simulink model "Dec_10_updated_33_bus_system_2MW_DG"  (R2023a)
settings: Solver=FixedStepAuto  StartTime=0.0  StopTime=0.3  RelTol=1e-3  EnableMultiTasking=on
undefined symbols (not defined in the file or in its folder): D1, Delta, DiscIntNeverNeededParam, Ts, Ts_Power
libraries: spsSeriesRLCBranchLib x42, spsThreePhaseVIMeasurementLib x35, spsThreePhaseSeriesRLCBranchLib x33, spsLoadFlowBusLib x33, spsThreePhaseParallelRLCLoadLib x31, simulink x8, spsMeanLib x5, spsFirstOrderFilterLib x4, spsStairGeneratorLib x3, spsBoostConverterLib x2, spsPowerPositiveSequenceLib x2, spsabctodq0Lib x2
(part 1 of 3)
settings Model: ExtModeTrigDuration=2  Creator=Archana  LastModifiedBy=praka
settings SolverCC: AutoInsertRateTranBlk=on
settings OptimizationCC: EnhancedBackFolding=on  PassReuseOutputArgsAs=Individual arguments  ZeroExternalMemoryAtStartup=off  ZeroInternalMemoryAtStartup=off  MaxStackSize=64  OptimizeBlockOrder=speed  DifferentSizesBufferReuse=on  OptimizationCustomize=off  EfficientTunableParamExpr=on
settings DebuggingCC: ParameterTunabilityLossMsg=error
settings HardwareCC: ProdBitPerPointer=32  ProdBitPerSizeT=32  ProdBitPerPtrDiffT=32  ProdLargestAtomicInteger=Long  ProdLargestAtomicFloat=Double  ProdWordSize=32  ProdHWDeviceType=ARM Compatible->ARM Cortex
settings SFSimCC: MATLABDynamicMemAlloc=off
settings RTWCC: Description=Embedded Coder  SystemTargetFile=ert.tlc  HardwareBoard=ESP32-WROVER(Arduino Compatible)  TLCOptions="-aInlineSetEventsForThisBaseRateFcn=TLC_FALSE -aSuppressMultiTaskScheduler=TLC_FALSE  -aRateBasedStepFcn=0"  TemplateMakefile=ert_default_tmf  Toolchain=ESP32  BuildConfiguration=Faster Runs
settings CodeAppCC: ForceParamTrailComments=on  IgnoreCustomStorageClasses=off  OperatorAnnotations=on  SimulinkDataObjDesc=on  SFDataObjDesc=on  InsertBlockDesc=on
settings ERTTargetCC: SupportContinuousTime=on  SupportVariableSizeSignals=on  ExtModeTransport=3  ExtModeStaticAlloc=on  ExtModeAutomaticAllocSize=off  ExtModeStaticAllocSize=65536  ExtModeMexFile=ext_xcp  ExtModeIntrfLevel=Level2 - Open

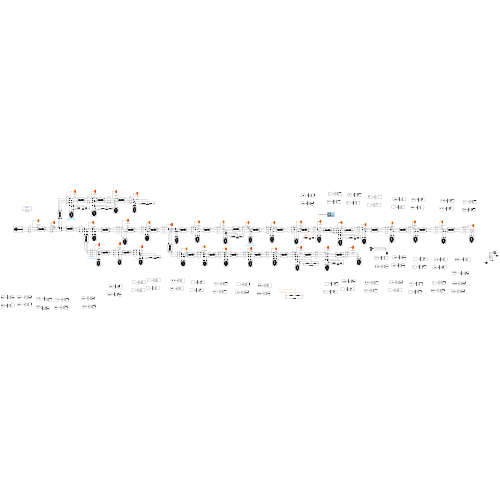
[thumbnail: Simulink's stored preview of the top-level diagram]
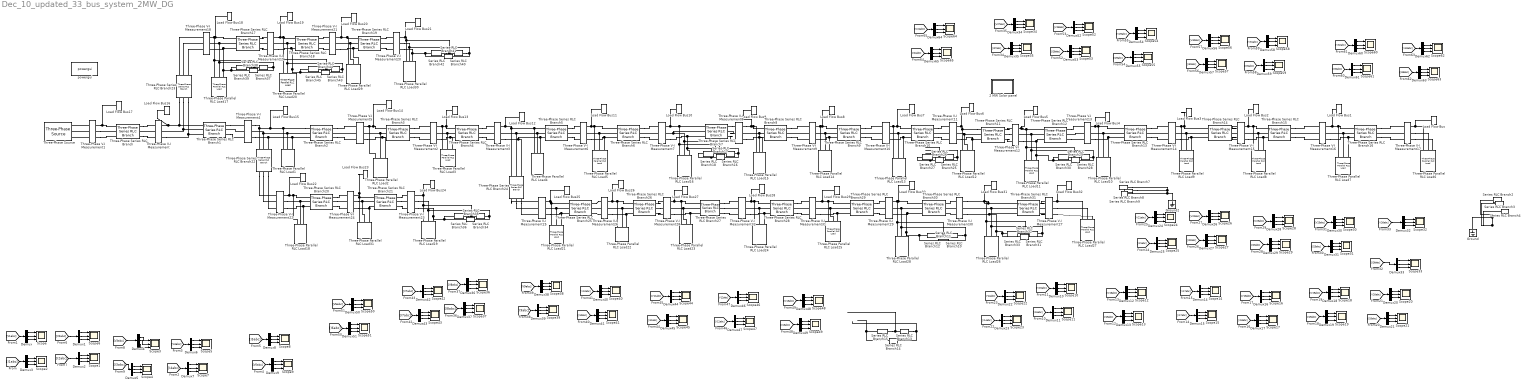
== system Dec_10_updated_33_bus_system_2MW_DG ==
  2 MW Solar panel : Subsystem
  Demux{,1..65} (66 alike) : Demux  Outputs=3
  Ground : spsGroundLib/Ground  LConnTagsString=a
  Ground2 : spsGroundLib/Ground  LConnTagsString=a
  Load Flow Bus : spsLoadFlowBusLib/Load Flow Bus  LConnTagsString=a  Phases=single  Connectors=on one side  ID=18  Vbase=12.66e3  Vref=1  Vangle=0  VLF=1  VLFb=1  VLFc=1  angleLF=0  angleLFb=0  angleLFc=0
  Load Flow Bus1 : spsLoadFlowBusLib/Load Flow Bus  LConnTagsString=a  Phases=single  Connectors=on one side  ID=17  Vbase=12.66e3  Vref=1  Vangle=0  VLF=1  VLFb=1  VLFc=1  angleLF=0  angleLFb=0  angleLFc=0
  Load Flow Bus10 : spsLoadFlowBusLib/Load Flow Bus  LConnTagsString=a  Phases=single  Connectors=on one side  ID=8  Vbase=12.66e3  Vref=1  Vangle=0  VLF=1  VLFb=1  VLFc=1  angleLF=0  angleLFb=0  angleLFc=0
  Load Flow Bus11 : spsLoadFlowBusLib/Load Flow Bus  LConnTagsString=a  Phases=single  Connectors=on one side  ID=7  Vbase=12.66e3  Vref=1  Vangle=0  VLF=1  VLFb=1  VLFc=1  angleLF=0  angleLFb=0  angleLFc=0
  Load Flow Bus12 : spsLoadFlowBusLib/Load Flow Bus  LConnTagsString=a  Phases=single  Connectors=on one side  ID=6  Vbase=12.66e3  Vref=1  Vangle=0  VLF=1  VLFb=1  VLFc=1  angleLF=0  angleLFb=0  angleLFc=0
  Load Flow Bus13 : spsLoadFlowBusLib/Load Flow Bus  LConnTagsString=a  Phases=single  Connectors=on one side  ID=5  Vbase=12.66e3  Vref=1  Vangle=0  VLF=1  VLFb=1  VLFc=1  angleLF=0  angleLFb=0  angleLFc=0
  Load Flow Bus14 : spsLoadFlowBusLib/Load Flow Bus  LConnTagsString=a  Phases=single  Connectors=on one side  ID=4  Vbase=12.66e3  Vref=1  Vangle=0  VLF=1  VLFb=1  VLFc=1  angleLF=0  angleLFb=0  angleLFc=0
  Load Flow Bus15 : spsLoadFlowBusLib/Load Flow Bus  LConnTagsString=a  Phases=single  Connectors=on one side  ID=3  Vbase=12.66e3  Vref=1  Vangle=0  VLF=1  VLFb=1  VLFc=1  angleLF=0  angleLFb=0  angleLFc=0
  Load Flow Bus16 : spsLoadFlowBusLib/Load Flow Bus  LConnTagsString=a  Phases=single  Connectors=on one side  ID=2  Vbase=12.66e3  Vref=1  Vangle=0  VLF=1  VLFb=1  VLFc=1  angleLF=0  angleLFb=0  angleLFc=0
  Load Flow Bus17 : spsLoadFlowBusLib/Load Flow Bus  LConnTagsString=a  Phases=single  Connectors=on one side  ID=1  Vbase=12.66e3  Vref=1.05  Vangle=0  VLF=1  VLFb=1  VLFc=1  angleLF=0  angleLFb=0  angleLFc=0
  Load Flow Bus18 : spsLoadFlowBusLib/Load Flow Bus  LConnTagsString=a  Phases=single  Connectors=on one side  ID=19  Vbase=12.66e3  Vref=1  Vangle=0  VLF=1  VLFb=1  VLFc=1  angleLF=0  angleLFb=0  angleLFc=0
  Load Flow Bus19 : spsLoadFlowBusLib/Load Flow Bus  LConnTagsString=a  Phases=single  Connectors=on one side  ID=20  Vbase=12.66e3  Vref=1  Vangle=0  VLF=1  VLFb=1  VLFc=1  angleLF=0  angleLFb=0  angleLFc=0
  Load Flow Bus2 : spsLoadFlowBusLib/Load Flow Bus  LConnTagsString=a  Phases=single  Connectors=on one side  ID=16  Vbase=12.66e3  Vref=1  Vangle=0  VLF=1  VLFb=1  VLFc=1  angleLF=0  angleLFb=0  angleLFc=0
  Load Flow Bus20 : spsLoadFlowBusLib/Load Flow Bus  LConnTagsString=a  Phases=single  Connectors=on one side  ID=21  Vbase=12.66e3  Vref=1  Vangle=0  VLF=1  VLFb=1  VLFc=1  angleLF=0  angleLFb=0  angleLFc=0
  Load Flow Bus21 : spsLoadFlowBusLib/Load Flow Bus  LConnTagsString=a  Phases=single  Connectors=on one side  ID=22  Vbase=12.66e3  Vref=1  Vangle=0  VLF=1  VLFb=1  VLFc=1  angleLF=0  angleLFb=0  angleLFc=0
  Load Flow Bus22 : spsLoadFlowBusLib/Load Flow Bus  LConnTagsString=a  Phases=single  Connectors=on one side  ID=23  Vbase=33e3  Vref=1  Vangle=0  VLF=1  VLFb=1  VLFc=1  angleLF=0  angleLFb=0  angleLFc=0
  Load Flow Bus23 : spsLoadFlowBusLib/Load Flow Bus  LConnTagsString=a  Phases=single  Connectors=on one side  ID=24  Vbase=33e3  Vref=1  Vangle=0  VLF=1  VLFb=1  VLFc=1  angleLF=0  angleLFb=0  angleLFc=0
  Load Flow Bus24 : spsLoadFlowBusLib/Load Flow Bus  LConnTagsString=a  Phases=single  Connectors=on one side  ID=25  Vbase=33e3  Vref=1  Vangle=0  VLF=1  VLFb=1  VLFc=1  angleLF=0  angleLFb=0  angleLFc=0
  Load Flow Bus25 : spsLoadFlowBusLib/Load Flow Bus  LConnTagsString=a  Phases=single  Connectors=on one side  ID=26  Vbase=12.66e3  Vref=1  Vangle=0  VLF=1  VLFb=1  VLFc=1  angleLF=0  angleLFb=0  angleLFc=0
  Load Flow Bus26 : spsLoadFlowBusLib/Load Flow Bus  LConnTagsString=a  Phases=single  Connectors=on one side  ID=27  Vbase=12.66e3  Vref=1  Vangle=0  VLF=1  VLFb=1  VLFc=1  angleLF=0  angleLFb=0  angleLFc=0
  Load Flow Bus27 : spsLoadFlowBusLib/Load Flow Bus  LConnTagsString=a  Phases=single  Connectors=on one side  ID=28  Vbase=12.66e3  Vref=1  Vangle=0  VLF=1  VLFb=1  VLFc=1  angleLF=0  angleLFb=0  angleLFc=0
  Load Flow Bus28 : spsLoadFlowBusLib/Load Flow Bus  LConnTagsString=a  Phases=single  Connectors=on one side  ID=29  Vbase=12.66e3  Vref=1  Vangle=0  VLF=1  VLFb=1  VLFc=1  angleLF=0  angleLFb=0  angleLFc=0
  Load Flow Bus29 : spsLoadFlowBusLib/Load Flow Bus  LConnTagsString=a  Phases=single  Connectors=on one side  ID=30  Vbase=12.66e3  Vref=1  Vangle=0  VLF=1  VLFb=1  VLFc=1  angleLF=0  angleLFb=0  angleLFc=0
  Load Flow Bus3 : spsLoadFlowBusLib/Load Flow Bus  LConnTagsString=a  Phases=single  Connectors=on one side  ID=15  Vbase=12.66e3  Vref=1  Vangle=0  VLF=1  VLFb=1  VLFc=1  angleLF=0  angleLFb=0  angleLFc=0
  Load Flow Bus30 : spsLoadFlowBusLib/Load Flow Bus  LConnTagsString=a  Phases=single  Connectors=on one side  ID=31  Vbase=12.66e3  Vref=1  Vangle=0  VLF=1  VLFb=1  VLFc=1  angleLF=0  angleLFb=0  angleLFc=0
  Load Flow Bus31 : spsLoadFlowBusLib/Load Flow Bus  LConnTagsString=a  Phases=single  Connectors=on one side  ID=32  Vbase=12.66e3  Vref=1  Vangle=0  VLF=1  VLFb=1  VLFc=1  angleLF=0  angleLFb=0  angleLFc=0
  Load Flow Bus32 : spsLoadFlowBusLib/Load Flow Bus  LConnTagsString=a  Phases=single  Connectors=on one side  ID=33  Vbase=12.66e3  Vref=1  Vangle=0  VLF=1  VLFb=1  VLFc=1  angleLF=0  angleLFb=0  angleLFc=0
  Load Flow Bus4 : spsLoadFlowBusLib/Load Flow Bus  LConnTagsString=a  Phases=single  Connectors=on one side  ID=14  Vbase=12.66e3  Vref=1  Vangle=0  VLF=1  VLFb=1  VLFc=1  angleLF=0  angleLFb=0  angleLFc=0
  Load Flow Bus5 : spsLoadFlowBusLib/Load Flow Bus  LConnTagsString=a  Phases=single  Connectors=on one side  ID=13  Vbase=12.66e3  Vref=1  Vangle=0  VLF=1  VLFb=1  VLFc=1  angleLF=0  angleLFb=0  angleLFc=0
  Load Flow Bus6 : spsLoadFlowBusLib/Load Flow Bus  LConnTagsString=a  Phases=single  Connectors=on one side  ID=12  Vbase=12.66e3  Vref=1  Vangle=0  VLF=1  VLFb=1  VLFc=1  angleLF=0  angleLFb=0  angleLFc=0
  Load Flow Bus7 : spsLoadFlowBusLib/Load Flow Bus  LConnTagsString=a  Phases=single  Connectors=on one side  ID=11  Vbase=12.66e3  Vref=1  Vangle=0  VLF=1  VLFb=1  VLFc=1  angleLF=0  angleLFb=0  angleLFc=0
  Load Flow Bus8 : spsLoadFlowBusLib/Load Flow Bus  LConnTagsString=a  Phases=single  Connectors=on one side  ID=10  Vbase=12.66e3  Vref=1  Vangle=0  VLF=1  VLFb=1  VLFc=1  angleLF=0  angleLFb=0  angleLFc=0
  Load Flow Bus9 : spsLoadFlowBusLib/Load Flow Bus  LConnTagsString=a  Phases=single  Connectors=on one side  ID=9  Vbase=12.66e3  Vref=1  Vangle=0  VLF=1  VLFb=1  VLFc=1  angleLF=0  angleLFb=0  angleLFc=0
  Scope{,1..65} (66 alike) : Scope  NumInputPorts=3
  Series RLC Branch10 : spsSeriesRLCBranchLib/Series RLC Branch  LConnTagsString=__new0  RConnTagsString=__new0  BranchType=C  Resistance=1  Inductance=0  SetiL0=off  InitialCurrent=0  Capacitance=4.53e-6  Setx0=off  InitialVoltage=0  Measurements=None
  Series RLC Branch11 : spsSeriesRLCBranchLib/Series RLC Branch  LConnTagsString=__new0  RConnTagsString=__new0  BranchType=C  Resistance=1  Inductance=0  SetiL0=off  InitialCurrent=0  Capacitance=4.53e-6  Setx0=off  InitialVoltage=0  Measurements=None
  Series RLC Branch12 : spsSeriesRLCBranchLib/Series RLC Branch  LConnTagsString=__new0  RConnTagsString=__new0  BranchType=C  Resistance=1  Inductance=0  SetiL0=off  InitialCurrent=0  Capacitance=4.53e-6  Setx0=off  InitialVoltage=0  Measurements=None
  Series RLC Branch13 : spsSeriesRLCBranchLib/Series RLC Branch  LConnTagsString=__new0  RConnTagsString=__new0  BranchType=C  Resistance=1  Inductance=0  SetiL0=off  InitialCurrent=0  Capacitance=0.144e-6  Setx0=off  InitialVoltage=0  Measurements=None
  Series RLC Branch14 : spsSeriesRLCBranchLib/Series RLC Branch  LConnTagsString=__new0  RConnTagsString=__new0  BranchType=C  Resistance=1  Inductance=0  SetiL0=off  InitialCurrent=0  Capacitance=0.144e-6  Setx0=off  InitialVoltage=0  Measurements=None
  Series RLC Branch15 : spsSeriesRLCBranchLib/Series RLC Branch  LConnTagsString=__new0  RConnTagsString=__new0  BranchType=C  Resistance=1  Inductance=0  SetiL0=off  InitialCurrent=0  Capacitance=0.144e-6  Setx0=off  InitialVoltage=0  Measurements=None
  Series RLC Branch16 : spsSeriesRLCBranchLib/Series RLC Branch  LConnTagsString=__new0  RConnTagsString=__new0  BranchType=C  Resistance=1  Inductance=0  SetiL0=off  InitialCurrent=0  Capacitance=1.44e-6  Setx0=off  InitialVoltage=0  Measurements=None
  Series RLC Branch17 : spsSeriesRLCBranchLib/Series RLC Branch  LConnTagsString=__new0  RConnTagsString=__new0  BranchType=C  Resistance=1  Inductance=0  SetiL0=off  InitialCurrent=0  Capacitance=1.44e-6  Setx0=off  InitialVoltage=0  Measurements=None
  Series RLC Branch18 : spsSeriesRLCBranchLib/Series RLC Branch  LConnTagsString=__new0  RConnTagsString=__new0  BranchType=C  Resistance=1  Inductance=0  SetiL0=off  InitialCurrent=0  Capacitance=1.44e-6  Setx0=off  InitialVoltage=0  Measurements=None
  Series RLC Branch2 : spsSeriesRLCBranchLib/Series RLC Branch  LConnTagsString=__new0  RConnTagsString=__new0  BranchType=C  Resistance=1  Inductance=0  SetiL0=off  InitialCurrent=0  Capacitance=3.26e-6  Setx0=off  InitialVoltage=0  Measurements=None
  Series RLC Branch25 : spsSeriesRLCBranchLib/Series RLC Branch  LConnTagsString=__new0  RConnTagsString=__new0  BranchType=C  Resistance=1  Inductance=0  SetiL0=off  InitialCurrent=0  Capacitance=0.755e-6  Setx0=off  InitialVoltage=0  Measurements=None
  Series RLC Branch26 : spsSeriesRLCBranchLib/Series RLC Branch  LConnTagsString=__new0  RConnTagsString=__new0  BranchType=C  Resistance=1  Inductance=0  SetiL0=off  InitialCurrent=0  Capacitance=0.755e-6  Setx0=off  InitialVoltage=0  Measurements=None
  Series RLC Branch27 : spsSeriesRLCBranchLib/Series RLC Branch  LConnTagsString=__new0  RConnTagsString=__new0  BranchType=C  Resistance=1  Inductance=0  SetiL0=off  InitialCurrent=0  Capacitance=0.755e-6  Setx0=off  InitialVoltage=0  Measurements=None
  Series RLC Branch28 : spsSeriesRLCBranchLib/Series RLC Branch  LConnTagsString=__new0  RConnTagsString=__new0  BranchType=C  Resistance=1  Inductance=0  SetiL0=off  InitialCurrent=0  Capacitance=0.594e-6  Setx0=off  InitialVoltage=0  Measurements=None
  Series RLC Branch29 : spsSeriesRLCBranchLib/Series RLC Branch  LConnTagsString=__new0  RConnTagsString=__new0  BranchType=C  Resistance=1  Inductance=0  SetiL0=off  InitialCurrent=0  Capacitance=0.594e-6  Setx0=off  InitialVoltage=0  Measurements=None
  Series RLC Branch3 : spsSeriesRLCBranchLib/Series RLC Branch  LConnTagsString=__new0  RConnTagsString=__new0  BranchType=C  Resistance=1  Inductance=0  SetiL0=off  InitialCurrent=0  Capacitance=3.26e-6  Setx0=off  InitialVoltage=0  Measurements=None
  Series RLC Branch30 : spsSeriesRLCBranchLib/Series RLC Branch  LConnTagsString=__new0  RConnTagsString=__new0  BranchType=C  Resistance=1  Inductance=0  SetiL0=off  InitialCurrent=0  Capacitance=0.594e-6  Setx0=off  InitialVoltage=0  Measurements=None
  Series RLC Branch31 : spsSeriesRLCBranchLib/Series RLC Branch  LConnTagsString=__new0  RConnTagsString=__new0  BranchType=C  Resistance=1  Inductance=0  SetiL0=off  InitialCurrent=0  Capacitance=0.472e-6  Setx0=off  InitialVoltage=0  Measurements=None
  Series RLC Branch32 : spsSeriesRLCBranchLib/Series RLC Branch  LConnTagsString=__new0  RConnTagsString=__new0  BranchType=C  Resistance=1  Inductance=0  SetiL0=off  InitialCurrent=0  Capacitance=0.472e-6  Setx0=off  InitialVoltage=0  Measurements=None
  Series RLC Branch33 : spsSeriesRLCBranchLib/Series RLC Branch  LConnTagsString=__new0  RConnTagsString=__new0  BranchType=C  Resistance=1  Inductance=0  SetiL0=off  InitialCurrent=0  Capacitance=0.472e-6  Setx0=off  InitialVoltage=0  Measurements=None
  Series RLC Branch34 : spsSeriesRLCBranchLib/Series RLC Branch  LConnTagsString=__new0  RConnTagsString=__new0  BranchType=C  Resistance=1  Inductance=0  SetiL0=off  InitialCurrent=0  Capacitance=0.614e-6  Setx0=off  InitialVoltage=0  Measurements=None
  Series RLC Branch35 : spsSeriesRLCBranchLib/Series RLC Branch  LConnTagsString=__new0  RConnTagsString=__new0  BranchType=C  Resistance=1  Inductance=0  SetiL0=off  InitialCurrent=0  Capacitance=0.614e-6  Setx0=off  InitialVoltage=0  Measurements=None
  Series RLC Branch36 : spsSeriesRLCBranchLib/Series RLC Branch  LConnTagsString=__new0  RConnTagsString=__new0  BranchType=C  Resistance=1  Inductance=0  SetiL0=off  InitialCurrent=0  Capacitance=0.614e-6  Setx0=off  InitialVoltage=0  Measurements=None
  Series RLC Branch37 : spsSeriesRLCBranchLib/Series RLC Branch  LConnTagsString=__new0  RConnTagsString=__new0  BranchType=C  Resistance=1  Inductance=0  SetiL0=off  InitialCurrent=0  Capacitance=0.434e-6  Setx0=off  InitialVoltage=0  Measurements=None
  Series RLC Branch38 : spsSeriesRLCBranchLib/Series RLC Branch  LConnTagsString=__new0  RConnTagsString=__new0  BranchType=C  Resistance=1  Inductance=0  SetiL0=off  InitialCurrent=0  Capacitance=0.434e-6  Setx0=off  InitialVoltage=0  Measurements=None
  Series RLC Branch39 : spsSeriesRLCBranchLib/Series RLC Branch  LConnTagsString=__new0  RConnTagsString=__new0  BranchType=C  Resistance=1  Inductance=0  SetiL0=off  InitialCurrent=0  Capacitance=0.434e-6  Setx0=off  InitialVoltage=0  Measurements=None
  Series RLC Branch4 : spsSeriesRLCBranchLib/Series RLC Branch  LConnTagsString=__new0  RConnTagsString=__new0  BranchType=C  Resistance=1  Inductance=0  SetiL0=off  InitialCurrent=0  Capacitance=3.26e-6  Setx0=off  InitialVoltage=0  Measurements=None
  Series RLC Branch40 : spsSeriesRLCBranchLib/Series RLC Branch  LConnTagsString=__new0  RConnTagsString=__new0  BranchType=C  Resistance=1  Inductance=0  SetiL0=off  InitialCurrent=0  Capacitance=0.107e-6  Setx0=off  InitialVoltage=0  Measurements=None
  Series RLC Branch41 : spsSeriesRLCBranchLib/Series RLC Branch  LConnTagsString=__new0  RConnTagsString=__new0  BranchType=C  Resistance=1  Inductance=0  SetiL0=off  InitialCurrent=0  Capacitance=0.107e-6  Setx0=off  InitialVoltage=0  Measurements=None
  Series RLC Branch42 : spsSeriesRLCBranchLib/Series RLC Branch  LConnTagsString=__new0  RConnTagsString=__new0  BranchType=C  Resistance=1  Inductance=0  SetiL0=off  InitialCurrent=0  Capacitance=0.107e-6  Setx0=off  InitialVoltage=0  Measurements=None
  Series RLC Branch43 : spsSeriesRLCBranchLib/Series RLC Branch  LConnTagsString=__new0  RConnTagsString=__new0  BranchType=C  Resistance=1  Inductance=0  SetiL0=off  InitialCurrent=0  Capacitance=0.322e-6  Setx0=off  InitialVoltage=0  Measurements=None
  Series RLC Branch44 : spsSeriesRLCBranchLib/Series RLC Branch  LConnTagsString=__new0  RConnTagsString=__new0  BranchType=C  Resistance=1  Inductance=0  SetiL0=off  InitialCurrent=0  Capacitance=0.322e-6  Setx0=off  InitialVoltage=0  Measurements=None
  Series RLC Branch45 : spsSeriesRLCBranchLib/Series RLC Branch  LConnTagsString=__new0  RConnTagsString=__new0  BranchType=C  Resistance=1  Inductance=0  SetiL0=off  InitialCurrent=0  Capacitance=0.322e-6  Setx0=off  InitialVoltage=0  Measurements=None
  Series RLC Branch7 : spsSeriesRLCBranchLib/Series RLC Branch  LConnTagsString=__new0  RConnTagsString=__new0  BranchType=C  Resistance=1  Inductance=0  SetiL0=off  InitialCurrent=0  Capacitance=36.8e-6  Setx0=off  InitialVoltage=0  Measurements=None
  Series RLC Branch8 : spsSeriesRLCBranchLib/Series RLC Branch  LConnTagsString=__new0  RConnTagsString=__new0  BranchType=C  Resistance=1  Inductance=0  SetiL0=off  InitialCurrent=0  Capacitance=36.8e-6  Setx0=off  InitialVoltage=0  Measurements=None
  Series RLC Branch9 : spsSeriesRLCBranchLib/Series RLC Branch  LConnTagsString=__new0  RConnTagsString=__new0  BranchType=C  Resistance=1  Inductance=0  SetiL0=off  InitialCurrent=0  Capacitance=36.8e-6  Setx0=off  InitialVoltage=0  Measurements=None
  Three-Phase Parallel RLC Load1 : spsThreePhaseParallelRLCLoadLib/Three-Phase Parallel RLC Load  LConnTagsString=A|B|C  Configuration=Y (grounded)  NominalVoltage=12.66e3  Vabc=[1e3 1e3 1e3]  Vabcp=[1e3 1e3 1e3]  NominalFrequency=50  UnbalancedPower=off  ActivePower=100e3  InductivePower=60e3  CapacitivePower=0  Pabc=[10e3 9e3 11e3]  QLabc=[100 90 110]  QCabc=[100 90 110]  Pabcp=[10e3 9e3 11e3]  QLabcp=[100 90 110]  QCabcp=[100 90 110]  Measurements=None  LoadType=constant PQ
  Three-Phase Parallel RLC Load10 : spsThreePhaseParallelRLCLoadLib/Three-Phase Parallel RLC Load  LConnTagsString=A|B|C  Configuration=Y (grounded)  NominalVoltage=12.66e3  Vabc=[1e3 1e3 1e3]  Vabcp=[1e3 1e3 1e3]  NominalFrequency=50  UnbalancedPower=off  ActivePower=60e3  InductivePower=35e3  CapacitivePower=0  Pabc=[10e3 9e3 11e3]  QLabc=[100 90 110]  QCabc=[100 90 110]  Pabcp=[10e3 9e3 11e3]  QLabcp=[100 90 110]  QCabcp=[100 90 110]  Measurements=None  LoadType=constant PQ
  Three-Phase Parallel RLC Load11 : spsThreePhaseParallelRLCLoadLib/Three-Phase Parallel RLC Load  LConnTagsString=A|B|C  Configuration=Y (grounded)  NominalVoltage=12.66e3  Vabc=[1e3 1e3 1e3]  Vabcp=[1e3 1e3 1e3]  NominalFrequency=50  UnbalancedPower=off  ActivePower=60e3  InductivePower=35e3  CapacitivePower=0  Pabc=[10e3 9e3 11e3]  QLabc=[100 90 110]  QCabc=[100 90 110]  Pabcp=[10e3 9e3 11e3]  QLabcp=[100 90 110]  QCabcp=[100 90 110]  Measurements=None  LoadType=constant PQ
  Three-Phase Parallel RLC Load12 : spsThreePhaseParallelRLCLoadLib/Three-Phase Parallel RLC Load  LConnTagsString=A|B|C  Configuration=Y (grounded)  NominalVoltage=12.66e3  Vabc=[1e3 1e3 1e3]  Vabcp=[1e3 1e3 1e3]  NominalFrequency=50  UnbalancedPower=off  ActivePower=45e3  InductivePower=30e3  CapacitivePower=0  Pabc=[10e3 9e3 11e3]  QLabc=[100 90 110]  QCabc=[100 90 110]  Pabcp=[10e3 9e3 11e3]  QLabcp=[100 90 110]  QCabcp=[100 90 110]  Measurements=None  LoadType=constant PQ
  Three-Phase Parallel RLC Load{5..7,13..14,24} (6 alike) : spsThreePhaseParallelRLCLoadLib/Three-Phase Parallel RLC Load  LConnTagsString=A|B|C  Configuration=Y (grounded)  NominalVoltage=12.66e3  Vabc=[1e3 1e3 1e3]  Vabcp=[1e3 1e3 1e3]  NominalFrequency=50  UnbalancedPower=off  ActivePower=60e3  InductivePower=20e3  CapacitivePower=0  Pabc=[10e3 9e3 11e3]  QLabc=[100 90 110]  QCabc=[100 90 110]  Pabcp=[10e3 9e3 11e3]  QLabcp=[100 90 110]  QCabcp=[100 90 110]  Measurements=None  LoadType=constant PQ
  Three-Phase Parallel RLC Load15 : spsThreePhaseParallelRLCLoadLib/Three-Phase Parallel RLC Load  LConnTagsString=A|B|C  Configuration=Y (grounded)  NominalVoltage=12.66e3  Vabc=[1e3 1e3 1e3]  Vabcp=[1e3 1e3 1e3]  NominalFrequency=50  UnbalancedPower=off  ActivePower=200e3  InductivePower=100e3  CapacitivePower=0  Pabc=[10e3 9e3 11e3]  QLabc=[100 90 110]  QCabc=[100 90 110]  Pabcp=[10e3 9e3 11e3]  QLabcp=[100 90 110]  QCabcp=[100 90 110]  Measurements=None  LoadType=constant PQ
  Three-Phase Parallel RLC Load16 : spsThreePhaseParallelRLCLoadLib/Three-Phase Parallel RLC Load  LConnTagsString=A|B|C  Configuration=Y (grounded)  NominalVoltage=12.66e3  Vabc=[1e3 1e3 1e3]  Vabcp=[1e3 1e3 1e3]  NominalFrequency=50  UnbalancedPower=off  ActivePower=200e3  InductivePower=100e3  CapacitivePower=0  Pabc=[10e3 9e3 11e3]  QLabc=[100 90 110]  QCabc=[100 90 110]  Pabcp=[10e3 9e3 11e3]  QLabcp=[100 90 110]  QCabcp=[100 90 110]  Measurements=None  LoadType=constant PQ
  Three-Phase Parallel RLC Load{2,17..18,20,29..30} (6 alike) : spsThreePhaseParallelRLCLoadLib/Three-Phase Parallel RLC Load  LConnTagsString=A|B|C  Configuration=Y (grounded)  NominalVoltage=12.66e3  Vabc=[1e3 1e3 1e3]  Vabcp=[1e3 1e3 1e3]  NominalFrequency=50  UnbalancedPower=off  ActivePower=90e3  InductivePower=40e3  CapacitivePower=0  Pabc=[10e3 9e3 11e3]  QLabc=[100 90 110]  QCabc=[100 90 110]  Pabcp=[10e3 9e3 11e3]  QLabcp=[100 90 110]  QCabcp=[100 90 110]  Measurements=None  LoadType=constant PQ
  Three-Phase Parallel RLC Load19 : spsThreePhaseParallelRLCLoadLib/Three-Phase Parallel RLC Load  LConnTagsString=A|B|C  Configuration=Y (grounded)  NominalVoltage=12.66e3  Vabc=[1e3 1e3 1e3]  Vabcp=[1e3 1e3 1e3]  NominalFrequency=50  UnbalancedPower=off  ActivePower=420e3  InductivePower=200e3  CapacitivePower=0  Pabc=[10e3 9e3 11e3]  QLabc=[100 90 110]  QCabc=[100 90 110]  Pabcp=[10e3 9e3 11e3]  QLabcp=[100 90 110]  QCabcp=[100 90 110]  Measurements=None  LoadType=constant PQ
  Three-Phase Parallel RLC Load21 : spsThreePhaseParallelRLCLoadLib/Three-Phase Parallel RLC Load  LConnTagsString=A|B|C  Configuration=Y (grounded)  NominalVoltage=12.66e3  Vabc=[1e3 1e3 1e3]  Vabcp=[1e3 1e3 1e3]  NominalFrequency=50  UnbalancedPower=off  ActivePower=420e3  InductivePower=200e3  CapacitivePower=0  Pabc=[10e3 9e3 11e3]  QLabc=[100 90 110]  QCabc=[100 90 110]  Pabcp=[10e3 9e3 11e3]  QLabcp=[100 90 110]  QCabcp=[100 90 110]  Measurements=None  LoadType=constant PQ
  Three-Phase Parallel RLC Load22 : spsThreePhaseParallelRLCLoadLib/Three-Phase Parallel RLC Load  LConnTagsString=A|B|C  Configuration=Y (grounded)  NominalVoltage=12.66e3  Vabc=[1e3 1e3 1e3]  Vabcp=[1e3 1e3 1e3]  NominalFrequency=50  UnbalancedPower=off  ActivePower=60e3  InductivePower=25e3  CapacitivePower=0  Pabc=[10e3 9e3 11e3]  QLabc=[100 90 110]  QCabc=[100 90 110]  Pabcp=[10e3 9e3 11e3]  QLabcp=[100 90 110]  QCabcp=[100 90 110]  Measurements=None  LoadType=constant PQ
  Three-Phase Parallel RLC Load23 : spsThreePhaseParallelRLCLoadLib/Three-Phase Parallel RLC Load  LConnTagsString=A|B|C  Configuration=Y (grounded)  NominalVoltage=12.66e3  Vabc=[1e3 1e3 1e3]  Vabcp=[1e3 1e3 1e3]  NominalFrequency=50  UnbalancedPower=off  ActivePower=60e3  InductivePower=25e3  CapacitivePower=0  Pabc=[10e3 9e3 11e3]  QLabc=[100 90 110]  QCabc=[100 90 110]  Pabcp=[10e3 9e3 11e3]  QLabcp=[100 90 110]  QCabcp=[100 90 110]  Measurements=None  LoadType=constant PQ
  Three-Phase Parallel RLC Load25 : spsThreePhaseParallelRLCLoadLib/Three-Phase Parallel RLC Load  LConnTagsString=A|B|C  Configuration=Y (grounded)  NominalVoltage=12.66e3  Vabc=[1e3 1e3 1e3]  Vabcp=[1e3 1e3 1e3]  NominalFrequency=50  UnbalancedPower=off  ActivePower=120e3  InductivePower=70e3  CapacitivePower=0  Pabc=[10e3 9e3 11e3]  QLabc=[100 90 110]  QCabc=[100 90 110]  Pabcp=[10e3 9e3 11e3]  QLabcp=[100 90 110]  QCabcp=[100 90 110]  Measurements=None  LoadType=constant PQ
  Three-Phase Parallel RLC Load26 : spsThreePhaseParallelRLCLoadLib/Three-Phase Parallel RLC Load  LConnTagsString=A|B|C  Configuration=Y (grounded)  NominalVoltage=12.66e3  Vabc=[1e3 1e3 1e3]  Vabcp=[1e3 1e3 1e3]  NominalFrequency=50  UnbalancedPower=off  ActivePower=150e3  InductivePower=70e3  CapacitivePower=0  Pabc=[10e3 9e3 11e3]  QLabc=[100 90 110]  QCabc=[100 90 110]  Pabcp=[10e3 9e3 11e3]  QLabcp=[100 90 110]  QCabcp=[100 90 110]  Measurements=None  LoadType=constant PQ
  Three-Phase Parallel RLC Load27 : spsThreePhaseParallelRLCLoadLib/Three-Phase Parallel RLC Load  LConnTagsString=A|B|C  Configuration=Y (grounded)  NominalVoltage=12.66e3  Vabc=[1e3 1e3 1e3]  Vabcp=[1e3 1e3 1e3]  NominalFrequency=50  UnbalancedPower=off  ActivePower=210e3  InductivePower=100e3  CapacitivePower=0  Pabc=[10e3 9e3 11e3]  QLabc=[100 90 110]  QCabc=[100 90 110]  Pabcp=[10e3 9e3 11e3]  QLabcp=[100 90 110]  QCabcp=[100 90 110]  Measurements=None  LoadType=constant PQ
  Three-Phase Parallel RLC Load28 : spsThreePhaseParallelRLCLoadLib/Three-Phase Parallel RLC Load  LConnTagsString=A|B|C  Configuration=Y (grounded)  NominalVoltage=12.66e3  Vabc=[1e3 1e3 1e3]  Vabcp=[1e3 1e3 1e3]  NominalFrequency=50  UnbalancedPower=off  ActivePower=200e3  InductivePower=600e3  CapacitivePower=0  Pabc=[10e3 9e3 11e3]  QLabc=[100 90 110]  QCabc=[100 90 110]  Pabcp=[10e3 9e3 11e3]  QLabcp=[100 90 110]  QCabcp=[100 90 110]  Measurements=None  LoadType=constant PQ
  Three-Phase Parallel RLC Load3 : spsThreePhaseParallelRLCLoadLib/Three-Phase Parallel RLC Load  LConnTagsString=A|B|C  Configuration=Y (grounded)  NominalVoltage=12.66e3  Vabc=[1e3 1e3 1e3]  Vabcp=[1e3 1e3 1e3]  NominalFrequency=50  UnbalancedPower=off  ActivePower=120e3  InductivePower=80e3  CapacitivePower=0  Pabc=[10e3 9e3 11e3]  QLabc=[100 90 110]  QCabc=[100 90 110]  Pabcp=[10e3 9e3 11e3]  QLabcp=[100 90 110]  QCabcp=[100 90 110]  Measurements=None  LoadType=constant PQ
  Three-Phase Parallel RLC Load31 : spsThreePhaseParallelRLCLoadLib/Three-Phase Parallel RLC Load  LConnTagsString=A|B|C  Configuration=Y (grounded)  NominalVoltage=12.66e3  Vabc=[1e3 1e3 1e3]  Vabcp=[1e3 1e3 1e3]  NominalFrequency=50  UnbalancedPower=off  ActivePower=90e3  InductivePower=50e3  CapacitivePower=0  Pabc=[10e3 9e3 11e3]  QLabc=[100 90 110]  QCabc=[100 90 110]  Pabcp=[10e3 9e3 11e3]  QLabcp=[100 90 110]  QCabcp=[100 90 110]  Measurements=None  LoadType=constant PQ
  Three-Phase Parallel RLC Load4 : spsThreePhaseParallelRLCLoadLib/Three-Phase Parallel RLC Load  LConnTagsString=A|B|C  Configuration=Y (grounded)  NominalVoltage=12.66e3  Vabc=[1e3 1e3 1e3]  Vabcp=[1e3 1e3 1e3]  NominalFrequency=50  UnbalancedPower=off  ActivePower=60e3  InductivePower=30e3  CapacitivePower=0  Pabc=[10e3 9e3 11e3]  QLabc=[100 90 110]  QCabc=[100 90 110]  Pabcp=[10e3 9e3 11e3]  QLabcp=[100 90 110]  QCabcp=[100 90 110]  Measurements=None  LoadType=constant PQ
  Three-Phase Parallel RLC Load8 : spsThreePhaseParallelRLCLoadLib/Three-Phase Parallel RLC Load  LConnTagsString=A|B|C  Configuration=Y (grounded)  NominalVoltage=12.66e3  Vabc=[1e3 1e3 1e3]  Vabcp=[1e3 1e3 1e3]  NominalFrequency=50  UnbalancedPower=off  ActivePower=60e3  InductivePower=10e3  CapacitivePower=0  Pabc=[10e3 9e3 11e3]  QLabc=[100 90 110]  QCabc=[100 90 110]  Pabcp=[10e3 9e3 11e3]  QLabcp=[100 90 110]  QCabcp=[100 90 110]  Measurements=None  LoadType=constant PQ
  Three-Phase Parallel RLC Load9 : spsThreePhaseParallelRLCLoadLib/Three-Phase Parallel RLC Load  LConnTagsString=A|B|C  Configuration=Y (grounded)  NominalVoltage=12.66e3  Vabc=[1e3 1e3 1e3]  Vabcp=[1e3 1e3 1e3]  NominalFrequency=50  UnbalancedPower=off  ActivePower=120e3  InductivePower=80e3  CapacitivePower=0  Pabc=[10e3 9e3 11e3]  QLabc=[100 90 110]  QCabc=[100 90 110]  Pabcp=[10e3 9e3 11e3]  QLabcp=[100 90 110]  QCabcp=[100 90 110]  Measurements=None  LoadType=constant PQ
  Three-Phase Series RLC Branch : spsThreePhaseSeriesRLCBranchLib/Three-Phase Series RLC Branch  LConnTagsString=A|B|C  RConnTagsString=A|B|C  BranchType=RL  Resistance=0.0922  Inductance=0.0477/314  Capacitance=1e-6  Measurements=None
  Three-Phase Series RLC Branch1 : spsThreePhaseSeriesRLCBranchLib/Three-Phase Series RLC Branch  LConnTagsString=A|B|C  RConnTagsString=A|B|C  BranchType=RL  Resistance=0.493  Inductance=0.2411/314  Capacitance=1e-6  Measurements=None
  Three-Phase Series RLC Branch10 : spsThreePhaseSeriesRLCBranchLib/Three-Phase Series RLC Branch  LConnTagsString=A|B|C  RConnTagsString=A|B|C  BranchType=RL  Resistance=0.3744  Inductance=0.1238/314  Capacitance=1e-6  Measurements=None
  Three-Phase Series RLC Branch11 : spsThreePhaseSeriesRLCBranchLib/Three-Phase Series RLC Branch  LConnTagsString=A|B|C  RConnTagsString=A|B|C  BranchType=RL  Resistance=1.468  Inductance=1.155/314  Capacitance=1e-6  Measurements=None
  Three-Phase Series RLC Branch12 : spsThreePhaseSeriesRLCBranchLib/Three-Phase Series RLC Branch  LConnTagsString=A|B|C  RConnTagsString=A|B|C  BranchType=RL  Resistance=0.5416  Inductance=0.7129/314  Capacitance=1e-6  Measurements=None
  Three-Phase Series RLC Branch13 : spsThreePhaseSeriesRLCBranchLib/Three-Phase Series RLC Branch  LConnTagsString=A|B|C  RConnTagsString=A|B|C  BranchType=RL  Resistance=0.591  Inductance=0.526/314  Capacitance=1e-6  Measurements=None
  Three-Phase Series RLC Branch14 : spsThreePhaseSeriesRLCBranchLib/Three-Phase Series RLC Branch  LConnTagsString=A|B|C  RConnTagsString=A|B|C  BranchType=RL  Resistance=0.7463  Inductance=0.545/314  Capacitance=1e-6  Measurements=None
  Three-Phase Series RLC Branch15 : spsThreePhaseSeriesRLCBranchLib/Three-Phase Series RLC Branch  LConnTagsString=A|B|C  RConnTagsString=A|B|C  BranchType=RL  Resistance=1.289  Inductance=1.721/314  Capacitance=1e-6  Measurements=None
  Three-Phase Series RLC Branch16 : spsThreePhaseSeriesRLCBranchLib/Three-Phase Series RLC Branch  LConnTagsString=A|B|C  RConnTagsString=A|B|C  BranchType=RL  Resistance=0.732  Inductance=0.574  Capacitance=1e-6  Measurements=None
  Three-Phase Series RLC Branch17 : spsThreePhaseSeriesRLCBranchLib/Three-Phase Series RLC Branch  LConnTagsString=A|B|C  RConnTagsString=A|B|C  BranchType=RL  Resistance=1.5042  Inductance=1.3554/314  Capacitance=1e-6  Measurements=None
  Three-Phase Series RLC Branch18 : spsThreePhaseSeriesRLCBranchLib/Three-Phase Series RLC Branch  LConnTagsString=A|B|C  RConnTagsString=A|B|C  BranchType=RL  Resistance=0.4095  Inductance=0.4784/314  Capacitance=1e-6  Measurements=None
  Three-Phase Series RLC Branch19 : spsThreePhaseSeriesRLCBranchLib/Three-Phase Series RLC Branch  LConnTagsString=A|B|C  RConnTagsString=A|B|C  BranchType=RL  Resistance=0.7089  Inductance=0.9373/314  Capacitance=1e-6  Measurements=None
  Three-Phase Series RLC Branch2 : spsThreePhaseSeriesRLCBranchLib/Three-Phase Series RLC Branch  LConnTagsString=A|B|C  RConnTagsString=A|B|C  BranchType=RL  Resistance=0.366  Inductance=0.1864/314  Capacitance=1e-6  Measurements=None
  Three-Phase Series RLC Branch20 : spsThreePhaseSeriesRLCBranchLib/Three-Phase Series RLC Branch  LConnTagsString=A|B|C  RConnTagsString=A|B|C  BranchType=RL  Resistance=0.898  Inductance=0.7091/314  Capacitance=1e-6  Measurements=None
  Three-Phase Series RLC Branch21 : spsThreePhaseSeriesRLCBranchLib/Three-Phase Series RLC Branch  LConnTagsString=A|B|C  RConnTagsString=A|B|C  BranchType=RL  Resistance=0.896  Inductance=0.7011/314  Capacitance=1e-6  Measurements=None
  Three-Phase Series RLC Branch22 : spsThreePhaseSeriesRLCBranchLib/Three-Phase Series RLC Branch  LConnTagsString=A|B|C  RConnTagsString=A|B|C  BranchType=RL  Resistance=0.4512  Inductance=0.3083/314  Capacitance=1e-6  Measurements=None
  Three-Phase Series RLC Branch23 : spsThreePhaseSeriesRLCBranchLib/Three-Phase Series RLC Branch  LConnTagsString=A|B|C  RConnTagsString=A|B|C  BranchType=RL  Resistance=0.164  Inductance=0.1565/314  Capacitance=1e-6  Measurements=None
  Three-Phase Series RLC Branch24 : spsThreePhaseSeriesRLCBranchLib/Three-Phase Series RLC Branch  LConnTagsString=A|B|C  RConnTagsString=A|B|C  BranchType=RL  Resistance=0.203  Inductance=0.1034/314  Capacitance=1e-6  Measurements=None
  Three-Phase Series RLC Branch25 : spsThreePhaseSeriesRLCBranchLib/Three-Phase Series RLC Branch  LConnTagsString=A|B|C  RConnTagsString=A|B|C  BranchType=RL  Resistance=0.2842  Inductance=0.1447/314  Capacitance=1e-6  Measurements=None
  Three-Phase Series RLC Branch26 : spsThreePhaseSeriesRLCBranchLib/Three-Phase Series RLC Branch  LConnTagsString=A|B|C  RConnTagsString=A|B|C  BranchType=RL  Resistance=1.0599  Inductance=0.9337/314  Capacitance=1e-6  Measurements=None
  Three-Phase Series RLC Branch27 : spsThreePhaseSeriesRLCBranchLib/Three-Phase Series RLC Branch  LConnTagsString=A|B|C  RConnTagsString=A|B|C  BranchType=RL  Resistance=0.8042  Inductance=0.7006/314  Capacitance=1e-6  Measurements=None
  Three-Phase Series RLC Branch28 : spsThreePhaseSeriesRLCBranchLib/Three-Phase Series RLC Branch  LConnTagsString=A|B|C  RConnTagsString=A|B|C  BranchType=RL  Resistance=0.5275  Inductance=0.2585/314  Capacitance=1e-6  Measurements=None
  Three-Phase Series RLC Branch29 : spsThreePhaseSeriesRLCBranchLib/Three-Phase Series RLC Branch  LConnTagsString=A|B|C  RConnTagsString=A|B|C  BranchType=RL  Resistance=0.9744  Inductance=0.963/314  Capacitance=1e-6  Measurements=None
  Three-Phase Series RLC Branch3 : spsThreePhaseSeriesRLCBranchLib/Three-Phase Series RLC Branch  LConnTagsString=A|B|C  RConnTagsString=A|B|C  BranchType=RL  Resistance=0.3811  Inductance=0.1941/314  Capacitance=1e-6  Measurements=None
  Three-Phase Series RLC Branch30 : spsThreePhaseSeriesRLCBranchLib/Three-Phase Series RLC Branch  LConnTagsString=A|B|C  RConnTagsString=A|B|C  BranchType=RL  Resistance=0.3105  Inductance=0.3619/314  Capacitance=1e-6  Measurements=None
  Three-Phase Series RLC Branch31 : spsThreePhaseSeriesRLCBranchLib/Three-Phase Series RLC Branch  LConnTagsString=A|B|C  RConnTagsString=A|B|C  BranchType=RL  Resistance=0.341  Inductance=0.5302/314  Capacitance=1e-6  Measurements=None
  Three-Phase Series RLC Branch4 : spsThreePhaseSeriesRLCBranchLib/Three-Phase Series RLC Branch  LConnTagsString=A|B|C  RConnTagsString=A|B|C  BranchType=RL  Resistance=0.8919  Inductance=0.707/314  Capacitance=1e-6  Measurements=None
  Three-Phase Series RLC Branch5 : spsThreePhaseSeriesRLCBranchLib/Three-Phase Series RLC Branch  LConnTagsString=A|B|C  RConnTagsString=A|B|C  BranchType=RL  Resistance=0.1872  Inductance=0.6188/314  Capacitance=1e-6  Measurements=None
  Three-Phase Series RLC Branch6 : spsThreePhaseSeriesRLCBranchLib/Three-Phase Series RLC Branch  LConnTagsString=A|B|C  RConnTagsString=A|B|C  BranchType=RL  Resistance=1.7114  Inductance=1.2351/314  Capacitance=1e-6  Measurements=None
  Three-Phase Series RLC Branch7 : spsThreePhaseSeriesRLCBranchLib/Three-Phase Series RLC Branch  LConnTagsString=A|B|C  RConnTagsString=A|B|C  BranchType=RL  Resistance=1.03  Inductance=0.74/314  Capacitance=1e-6  Measurements=None
  Three-Phase Series RLC Branch8 : spsThreePhaseSeriesRLCBranchLib/Three-Phase Series RLC Branch  LConnTagsString=A|B|C  RConnTagsString=A|B|C  BranchType=RL  Resistance=1.04  Inductance=0.74/314  Capacitance=1e-6  Measurements=None
  Three-Phase Series RLC Branch9 : spsThreePhaseSeriesRLCBranchLib/Three-Phase Series RLC Branch  LConnTagsString=A|B|C  RConnTagsString=A|B|C  BranchType=RL  Resistance=0.1966  Inductance=0.065/314  Capacitance=1e-6  Measurements=None
  Three-Phase V-I Measurement : spsThreePhaseVIMeasurementLib/Three-Phase V-I Measurement  VoltageMeasurement=phase-to-ground  SetLabelV=on  LabelV=V2abc  Vpu=off  VpuLL=off  CurrentMeasurement=yes  SetLabelI=on  LabelI=I2abc  Ipu=off  Pbase=100e6  Vbase=500e3  OutputType=Complex  PhasorSimulation=off  PSBequivalent=0
  Three-Phase V-I Measurement1 : spsThreePhaseVIMeasurementLib/Three-Phase V-I Measurement  VoltageMeasurement=phase-to-ground  SetLabelV=on  LabelV=V1abc  Vpu=off  VpuLL=off  CurrentMeasurement=yes  SetLabelI=on  LabelI=I1abc  Ipu=off  Pbase=100e6  Vbase=500e3  OutputType=Complex  PhasorSimulation=off  PSBequivalent=0
  Three-Phase V-I Measurement10 : spsThreePhaseVIMeasurementLib/Three-Phase V-I Measurement  VoltageMeasurement=phase-to-ground  SetLabelV=on  LabelV=V11abc  Vpu=off  VpuLL=off  CurrentMeasurement=yes  SetLabelI=on  LabelI=I11abc  Ipu=off  Pbase=100e6  Vbase=500e3  OutputType=Complex  PhasorSimulation=off  PSBequivalent=0
  Three-Phase V-I Measurement11 : spsThreePhaseVIMeasurementLib/Three-Phase V-I Measurement  VoltageMeasurement=phase-to-ground  SetLabelV=on  LabelV=V12abc  Vpu=off  VpuLL=off  CurrentMeasurement=yes  SetLabelI=on  LabelI=I12abc  Ipu=off  Pbase=100e6  Vbase=500e3  OutputType=Complex  PhasorSimulation=off  PSBequivalent=0
  Three-Phase V-I Measurement12 : spsThreePhaseVIMeasurementLib/Three-Phase V-I Measurement  VoltageMeasurement=phase-to-ground  SetLabelV=on  LabelV=V13abc  Vpu=off  VpuLL=off  CurrentMeasurement=yes  SetLabelI=on  LabelI=I13abc  Ipu=off  Pbase=100e6  Vbase=500e3  OutputType=Complex  PhasorSimulation=off  PSBequivalent=0
  Three-Phase V-I Measurement13 : spsThreePhaseVIMeasurementLib/Three-Phase V-I Measurement  VoltageMeasurement=phase-to-ground  SetLabelV=on  LabelV=V14abc  Vpu=off  VpuLL=off  CurrentMeasurement=yes  SetLabelI=on  LabelI=I14abc  Ipu=off  Pbase=100e6  Vbase=500e3  OutputType=Complex  PhasorSimulation=off  PSBequivalent=0
  Three-Phase V-I Measurement14 : spsThreePhaseVIMeasurementLib/Three-Phase V-I Measurement  VoltageMeasurement=phase-to-ground  SetLabelV=on  LabelV=V15abc  Vpu=off  VpuLL=off  CurrentMeasurement=yes  SetLabelI=on  LabelI=I15abc  Ipu=off  Pbase=100e6  Vbase=500e3  OutputType=Complex  PhasorSimulation=off  PSBequivalent=0
  Three-Phase V-I Measurement15 : spsThreePhaseVIMeasurementLib/Three-Phase V-I Measurement  VoltageMeasurement=phase-to-ground  SetLabelV=on  LabelV=V16abc  Vpu=off  VpuLL=off  CurrentMeasurement=yes  SetLabelI=on  LabelI=I16abc  Ipu=off  Pbase=100e6  Vbase=500e3  OutputType=Complex  PhasorSimulation=off  PSBequivalent=0
  Three-Phase V-I Measurement16 : spsThreePhaseVIMeasurementLib/Three-Phase V-I Measurement  VoltageMeasurement=phase-to-ground  SetLabelV=on  LabelV=V17abc  Vpu=off  VpuLL=off  CurrentMeasurement=yes  SetLabelI=on  LabelI=I17abc  Ipu=off  Pbase=100e6  Vbase=500e3  OutputType=Complex  PhasorSimulation=off  PSBequivalent=0
  Three-Phase V-I Measurement17 : spsThreePhaseVIMeasurementLib/Three-Phase V-I Measurement  VoltageMeasurement=phase-to-ground  SetLabelV=on  LabelV=V18abc  Vpu=off  VpuLL=off  CurrentMeasurement=yes  SetLabelI=on  LabelI=I18abc  Ipu=off  Pbase=100e6  Vbase=500e3  OutputType=Complex  PhasorSimulation=off  PSBequivalent=0
  Three-Phase V-I Measurement18 : spsThreePhaseVIMeasurementLib/Three-Phase V-I Measurement  VoltageMeasurement=phase-to-ground  SetLabelV=on  LabelV=V19abc  Vpu=off  VpuLL=off  CurrentMeasurement=yes  SetLabelI=on  LabelI=I19abc  Ipu=off  Pbase=100e6  Vbase=500e3  OutputType=Complex  PhasorSimulation=off  PSBequivalent=0
  Three-Phase V-I Measurement19 : spsThreePhaseVIMeasurementLib/Three-Phase V-I Measurement  VoltageMeasurement=phase-to-ground  SetLabelV=on  LabelV=V20abc  Vpu=off  VpuLL=off  CurrentMeasurement=yes  SetLabelI=on  LabelI=I20abc  Ipu=off  Pbase=100e6  Vbase=500e3  OutputType=Complex  PhasorSimulation=off  PSBequivalent=0
  Three-Phase V-I Measurement2 : spsThreePhaseVIMeasurementLib/Three-Phase V-I Measurement  VoltageMeasurement=phase-to-ground  SetLabelV=on  LabelV=V5abc  Vpu=off  VpuLL=off  CurrentMeasurement=yes  SetLabelI=on  LabelI=I5abc  Ipu=off  Pbase=100e6  Vbase=500e3  OutputType=Complex  PhasorSimulation=off  PSBequivalent=0
  Three-Phase V-I Measurement20 : spsThreePhaseVIMeasurementLib/Three-Phase V-I Measurement  VoltageMeasurement=phase-to-ground  SetLabelV=on  LabelV=V22abc  Vpu=off  VpuLL=off  CurrentMeasurement=yes  SetLabelI=on  LabelI=I22abc  Ipu=off  Pbase=100e6  Vbase=500e3  OutputType=Complex  PhasorSimulation=off  PSBequivalent=0
  Three-Phase V-I Measurement21 : spsThreePhaseVIMeasurementLib/Three-Phase V-I Measurement  VoltageMeasurement=phase-to-ground  SetLabelV=on  LabelV=V21abc  Vpu=off  VpuLL=off  CurrentMeasurement=yes  SetLabelI=on  LabelI=I21abc  Ipu=off  Pbase=100e6  Vbase=500e3  OutputType=Complex  PhasorSimulation=off  PSBequivalent=0
  Three-Phase V-I Measurement22 : spsThreePhaseVIMeasurementLib/Three-Phase V-I Measurement  VoltageMeasurement=phase-to-ground  SetLabelV=on  LabelV=V23abc  Vpu=off  VpuLL=off  CurrentMeasurement=yes  SetLabelI=on  LabelI=I23abc  Ipu=off  Pbase=100e6  Vbase=500e3  OutputType=Complex  PhasorSimulation=off  PSBequivalent=0
  Three-Phase V-I Measurement23 : spsThreePhaseVIMeasurementLib/Three-Phase V-I Measurement  VoltageMeasurement=phase-to-ground  SetLabelV=on  LabelV=V25abc  Vpu=off  VpuLL=off  CurrentMeasurement=yes  SetLabelI=on  LabelI=I25abc  Ipu=off  Pbase=100e6  Vbase=500e3  OutputType=Complex  PhasorSimulation=off  PSBequivalent=0
  Three-Phase V-I Measurement24 : spsThreePhaseVIMeasurementLib/Three-Phase V-I Measurement  VoltageMeasurement=phase-to-ground  SetLabelV=on  LabelV=V24abc  Vpu=off  VpuLL=off  CurrentMeasurement=yes  SetLabelI=on  LabelI=I24abc  Ipu=off  Pbase=100e6  Vbase=500e3  OutputType=Complex  PhasorSimulation=off  PSBequivalent=0
  Three-Phase V-I Measurement25 : spsThreePhaseVIMeasurementLib/Three-Phase V-I Measurement  VoltageMeasurement=phase-to-ground  SetLabelV=on  LabelV=V26abc  Vpu=off  VpuLL=off  CurrentMeasurement=yes  SetLabelI=on  LabelI=I26abc  Ipu=off  Pbase=100e6  Vbase=500e3  OutputType=Complex  PhasorSimulation=off  PSBequivalent=0
  Three-Phase V-I Measurement26 : spsThreePhaseVIMeasurementLib/Three-Phase V-I Measurement  VoltageMeasurement=phase-to-ground  SetLabelV=on  LabelV=V27abc  Vpu=off  VpuLL=off  CurrentMeasurement=yes  SetLabelI=on  LabelI=I27abc  Ipu=off  Pbase=100e6  Vbase=500e3  OutputType=Complex  PhasorSimulation=off  PSBequivalent=0
  Three-Phase V-I Measurement27 : spsThreePhaseVIMeasurementLib/Three-Phase V-I Measurement  VoltageMeasurement=phase-to-ground  SetLabelV=on  LabelV=V33abc  Vpu=off  VpuLL=off  CurrentMeasurement=yes  SetLabelI=on  LabelI=I33abc  Ipu=off  Pbase=100e6  Vbase=500e3  OutputType=Complex  PhasorSimulation=off  PSBequivalent=0
  Three-Phase V-I Measurement28 : spsThreePhaseVIMeasurementLib/Three-Phase V-I Measurement  VoltageMeasurement=phase-to-ground  SetLabelV=on  LabelV=V28abc  Vpu=off  VpuLL=off  CurrentMeasurement=yes  SetLabelI=on  LabelI=I28abc  Ipu=off  Pbase=100e6  Vbase=500e3  OutputType=Complex  PhasorSimulation=off  PSBequivalent=0
  Three-Phase V-I Measurement29 : spsThreePhaseVIMeasurementLib/Three-Phase V-I Measurement  VoltageMeasurement=phase-to-ground  SetLabelV=on  LabelV=V31abc  Vpu=off  VpuLL=off  CurrentMeasurement=yes  SetLabelI=on  LabelI=I31abc  Ipu=off  Pbase=100e6  Vbase=500e3  OutputType=Complex  PhasorSimulation=off  PSBequivalent=0
  Three-Phase V-I Measurement3 : spsThreePhaseVIMeasurementLib/Three-Phase V-I Measurement  VoltageMeasurement=phase-to-ground  SetLabelV=on  LabelV=V6abc  Vpu=off  VpuLL=off  CurrentMeasurement=yes  SetLabelI=on  LabelI=I6abc  Ipu=off  Pbase=100e6  Vbase=500e3  OutputType=Complex  PhasorSimulation=off  PSBequivalent=0
  Three-Phase V-I Measurement30 : spsThreePhaseVIMeasurementLib/Three-Phase V-I Measurement  VoltageMeasurement=phase-to-ground  SetLabelV=on  LabelV=V32abc  Vpu=off  VpuLL=off  CurrentMeasurement=yes  SetLabelI=on  LabelI=I32abc  Ipu=off  Pbase=100e6  Vbase=500e3  OutputType=Complex  PhasorSimulation=off  PSBequivalent=0
  Three-Phase V-I Measurement31 : spsThreePhaseVIMeasurementLib/Three-Phase V-I Measurement  VoltageMeasurement=phase-to-ground  SetLabelV=on  LabelV=V30abc  Vpu=off  VpuLL=off  CurrentMeasurement=yes  SetLabelI=on  LabelI=I30abc  Ipu=off  Pbase=100e6  Vbase=500e3  OutputType=Complex  PhasorSimulation=off  PSBequivalent=0
  Three-Phase V-I Measurement32 : spsThreePhaseVIMeasurementLib/Three-Phase V-I Measurement  VoltageMeasurement=phase-to-ground  SetLabelV=on  LabelV=V29abc  Vpu=off  VpuLL=off  CurrentMeasurement=yes  SetLabelI=on  LabelI=I29abc  Ipu=off  Pbase=100e6  Vbase=500e3  OutputType=Complex  PhasorSimulation=off  PSBequivalent=0
  Three-Phase V-I Measurement4 : spsThreePhaseVIMeasurementLib/Three-Phase V-I Measurement  VoltageMeasurement=phase-to-ground  SetLabelV=on  LabelV=V3abc  Vpu=off  VpuLL=off  CurrentMeasurement=yes  SetLabelI=on  LabelI=I3abc  Ipu=off  Pbase=100e6  Vbase=500e3  OutputType=Complex  PhasorSimulation=off  PSBequivalent=0
  Three-Phase V-I Measurement5 : spsThreePhaseVIMeasurementLib/Three-Phase V-I Measurement  VoltageMeasurement=phase-to-ground  SetLabelV=on  LabelV=V4abc  Vpu=off  VpuLL=off  CurrentMeasurement=yes  SetLabelI=on  LabelI=I4abc  Ipu=off  Pbase=100e6  Vbase=500e3  OutputType=Complex  PhasorSimulation=off  PSBequivalent=0
  Three-Phase V-I Measurement6 : spsThreePhaseVIMeasurementLib/Three-Phase V-I Measurement  VoltageMeasurement=phase-to-ground  SetLabelV=on  LabelV=V7abc  Vpu=off  VpuLL=off  CurrentMeasurement=yes  SetLabelI=on  LabelI=I7abc  Ipu=off  Pbase=100e6  Vbase=500e3  OutputType=Complex  PhasorSimulation=off  PSBequivalent=0
  Three-Phase V-I Measurement7 : spsThreePhaseVIMeasurementLib/Three-Phase V-I Measurement  VoltageMeasurement=phase-to-ground  SetLabelV=on  LabelV=V8abc  Vpu=off  VpuLL=off  CurrentMeasurement=yes  SetLabelI=on  LabelI=I8abc  Ipu=off  Pbase=100e6  Vbase=500e3  OutputType=Complex  PhasorSimulation=off  PSBequivalent=0
  Three-Phase V-I Measurement8 : spsThreePhaseVIMeasurementLib/Three-Phase V-I Measurement  VoltageMeasurement=phase-to-ground  SetLabelV=on  LabelV=V9abc  Vpu=off  VpuLL=off  CurrentMeasurement=yes  SetLabelI=on  LabelI=I9abc  Ipu=off  Pbase=100e6  Vbase=500e3  OutputType=Complex  PhasorSimulation=off  PSBequivalent=0
  Three-Phase V-I Measurement9 : spsThreePhaseVIMeasurementLib/Three-Phase V-I Measurement  VoltageMeasurement=phase-to-ground  SetLabelV=on  LabelV=V10abc  Vpu=off  VpuLL=off  CurrentMeasurement=yes  SetLabelI=on  LabelI=I10abc  Ipu=off  Pbase=100e6  Vbase=500e3  OutputType=Complex  PhasorSimulation=off  PSBequivalent=0
  Three-Phase Source : spsThreePhaseSourceLib/Three-Phase Source  InternalConnection=Yg  VoltagePhases=off  Voltage=12.66e3*1.05  PhaseAngle=0  Voltage_phases=[25e3 25e3 25e3]/sqrt(3)  PhaseAngles_phases=[0 -120 +120]  Frequency=50  NonIdealSource=on  SpecifyImpedance=off  Resistance=0  Inductance=0  ShortCircuitLevel=100e6  BaseVoltage=12.66e3  XRratio=7  BusType=swing  Pref=10e3  Qref=0  Prefabc=[10e3, 10e3, 10e3]  Qrefabc=[0, 0, 0]  Qmin=-inf  Qmax=inf
  powergui : spspowerguiLib/powergui  Priority=1  SimulationMode=Discrete  SampleTime=1e-6  frequency=60  Iterations=50  frequencyindice=50  Pbase=100e6  ErrMax=1e-4  UnitsV=kV  UnitsW=MW  buscounter=0  FunctionMessages=off  echomessages=off  EnableUseOfTLC=off  CurrentSourceSwitches=off  DisableSnubberDevices=off  DisableRonSwitches=off  DisableVfSwitches=off  DisplayEquations=off  AutomaticDiscreteSolvers=off  SolverType=Tustin/Backward Euler (TBE)  Interpol=off  ExternalGateDelay=off  methode=off  Ts=100  x0status=blocks  SPID=on  SwTol=0  HookPort=off  NonlinearTolerance=1e-4  nMaxIteration=100  ContinueOnMaxIteration=off  RestoreLinks=warning  ResistiveCurrentMeasurement=off  Frange=[0:2:500]  Ylog=off  Xlog=on  ShowGrid=off  save=off  variable=ZData  structure=0  ZoomFFT=off  StartTime=0.0  cycles=1  DisplayStyle=1  fundamental=60  FreqAxis=off  MaxFrequency=1000  frequencyindicesteady=1  RmsSteady=1  display=off
  wires:
  Demux65/1 -> Scope65/1
  Demux65/3 -> Scope65/3
  [I24abc] -> Demux65/1
  [I28abc] -> Demux53/1
  Demux53/2 -> Scope53/2
  Demux52/1 -> Scope52/1
  Demux52/2 -> Scope52/2
  Demux53/1 -> Scope53/1
  Demux58/1 -> Scope58/1
  Demux59/2 -> Scope59/2
  [V31abc] -> Demux58/1
  Demux35/2 -> Scope35/2
  [I27abc] -> Demux35/1
  Demux35/3 -> Scope35/3
  Demux34/2 -> Scope34/2
  Demux34/1 -> Scope34/1
  Demux52/3 -> Scope52/3
  Demux34/3 -> Scope34/3
  [V24abc] -> Demux64/1
  [V32abc] -> Demux60/1
  Demux61/2 -> Scope61/2
  Demux60/1 -> Scope60/1
  Demux61/1 -> Scope61/1
  Demux60/3 -> Scope60/3
  Demux60/2 -> Scope60/2
  Demux38/1 -> Scope38/1
  [I9abc] -> Demux39/1
  Demux39/1 -> Scope39/1
  Demux38/3 -> Scope38/3
  [I8abc] -> Demux37/1
  Demux37/3 -> Scope37/3
  [V8abc] -> Demux36/1
  Demux42/3 -> Scope42/3
  [I7abc] -> Demux43/1
  Demux43/1 -> Scope43/1
  Demux42/1 -> Scope42/1
  Demux43/3 -> Scope43/3
  Demux48/1 -> Scope48/1
  [V13abc] -> Demux48/1
  [I13abc] -> Demux49/1
  Demux49/1 -> Scope49/1
  [I16abc] -> Demux13/1
  Demux13/1 -> Scope13/1
  Demux12/3 -> Scope12/3
  [V10abc] -> Demux40/1
  Demux48/2 -> Scope48/2
  Demux40/1 -> Scope40/1
  Demux12/1 -> Scope12/1
  [I10abc] -> Demux41/1
  Demux41/2 -> Scope41/2
  Demux13/3 -> Scope13/3
  [I22abc] -> Demux27/1
  Demux27/2 -> Scope27/2
  Demux27/3 -> Scope27/3
  Demux19/2 -> Scope19/2
  Demux19/3 -> Scope19/3
  Demux18/1 -> Scope18/1
  Demux18/2 -> Scope18/2
  [I14abc] -> Demux23/1
  Demux23/2 -> Scope23/2
  [V14abc] -> Demux22/1
  Demux23/3 -> Scope23/3
  Demux22/1 -> Scope22/1
  Demux22/2 -> Scope22/2
  [I11abc] -> Demux45/1
  Demux45/1 -> Scope45/1
  Demux44/1 -> Scope44/1
  [I12abc] -> Demux47/1
  Demux37/2 -> Scope37/2
  [V12abc] -> Demux46/1
  Demux46/1 -> Scope46/1
  Demux46/3 -> Scope46/3
  Demux46/2 -> Scope46/2
  [I18abc] -> Demux17/1
  Demux16/2 -> Scope16/2
  Demux49/3 -> Scope49/3
  Demux17/3 -> Scope17/3
  Demux17/2 -> Scope17/2
  Demux17/1 -> Scope17/1
  [V27abc] -> Demux34/1
  Demux16/3 -> Scope16/3
  [V15abc] -> Demux10/1
  Demux11/2 -> Scope11/2
  [I15abc] -> Demux11/1
  Demux10/3 -> Scope10/3
  Demux11/1 -> Scope11/1
  Demux33/2 -> Scope33/2
  Demux32/1 -> Scope32/1
  [V26abc] -> Demux32/1
  Demux33/3 -> Scope33/3
  Demux33/1 -> Scope33/1
  Demux32/2 -> Scope32/2
  [V17abc] -> Demux14/1
  Demux14/1 -> Scope14/1
  Demux40/3 -> Scope40/3
  Demux15/1 -> Scope15/1
  Demux15/3 -> Scope15/3
  Demux14/3 -> Scope14/3
  Demux14/2 -> Scope14/2
  Demux21/3 -> Scope21/3
  [V19abc] -> Demux18/1
  Demux20/3 -> Scope20/3
  Demux21/2 -> Scope21/2
  Demux12/2 -> Scope12/2
  [V20abc] -> Demux20/1
  Demux20/2 -> Scope20/2
  Demux55/2 -> Scope55/2
  Demux55/3 -> Scope55/3
  Demux54/1 -> Scope54/1
  Demux26/2 -> Scope26/2
  [I29abc] -> Demux55/1
  [V29abc] -> Demux54/1
  Demux54/2 -> Scope54/2
  [I25abc] -> Demux31/1
  Demux30/2 -> Scope30/2
  Demux30/1 -> Scope30/1
  Demux31/1 -> Scope31/1
  Demux30/3 -> Scope30/3
  Demux29/2 -> Scope29/2
  Demux29/1 -> Scope29/1
  Demux28/3 -> Scope28/3
  Demux51/2 -> Scope51/2
  Demux50/3 -> Scope50/3
  Demux51/3 -> Scope51/3
  Demux57/3 -> Scope57/3
  Demux59/1 -> Scope59/1
  Demux56/1 -> Scope56/1
  Demux56/3 -> Scope56/3
  Demux24/1 -> Scope24/1
  Demux24/3 -> Scope24/3
  Demux25/2 -> Scope25/2
  Demux25/1 -> Scope25/1
  Demux10/2 -> Scope10/2
  Demux62/1 -> Scope62/1
  [V33abc] -> Demux62/1
  Demux59/3 -> Scope59/3
  Demux63/3 -> Scope63/3
  [V21abc] -> Demux24/1
  [I4abc] -> Demux7/1
  Demux1/3 -> Scope6/3
  [I1abc] -> Demux3/1
  [V30abc] -> Demux56/1
  Demux13/2 -> Scope13/2
  Demux47/1 -> Scope47/1
  Demux45/2 -> Scope45/2
  Demux36/3 -> Scope36/3
  Demux62/3 -> Scope62/3
  Demux47/2 -> Scope47/2
  Demux29/3 -> Scope29/3
  Demux48/3 -> Scope48/3
  Demux53/3 -> Scope53/3
  Demux56/2 -> Scope56/2
  Demux57/2 -> Scope57/2
  Demux36/1 -> Scope36/1
  Demux50/2 -> Scope50/2
  Demux/3 -> Scope/3
  Demux24/2 -> Scope24/2
  Demux20/1 -> Scope20/1
  Demux31/3 -> Scope31/3
  Demux44/2 -> Scope44/2
  Demux18/3 -> Scope18/3
  [I3abc] -> Demux5/1
  Demux58/3 -> Scope58/3
  [I32abc] -> Demux61/1
  Demux38/2 -> Scope38/2
  Demux40/2 -> Scope40/2
  Demux35/1 -> Scope35/1
  Demux4/3 -> Scope3/3
  Demux/1 -> Scope/1
  Demux10/1 -> Scope10/1
  Demux51/1 -> Scope51/1
  Demux22/3 -> Scope22/3
  Demux9/2 -> Scope9/2
  Demux6/2 -> Scope5/2
  [V6abc] -> Demux50/1
  Demux26/1 -> Scope26/1
  [I5abc] -> Demux8/1
  Demux42/2 -> Scope42/2
  Demux27/1 -> Scope27/1
  [V28abc] -> Demux52/1
  [I6abc] -> Demux51/1
  Demux44/3 -> Scope44/3
  Demux26/3 -> Scope26/3
  [V11abc] -> Demux44/1
  [V23abc] -> Demux28/1
  Demux54/3 -> Scope54/3
  Demux28/2 -> Scope28/2
  Demux31/2 -> Scope31/2
  Demux64/1 -> Scope64/1
  Demux28/1 -> Scope28/1
  [I23abc] -> Demux29/1
  [I20abc] -> Demux21/1
  Demux9/3 -> Scope9/3
  Demux39/2 -> Scope39/2
  Demux47/3 -> Scope47/3
  Demux25/3 -> Scope25/3
  Demux36/2 -> Scope36/2
  Demux37/1 -> Scope37/1
  Demux63/1 -> Scope63/1
  Demux39/3 -> Scope39/3
  Demux11/3 -> Scope11/3
  [V3abc] -> Demux4/1
  Demux63/2 -> Scope63/2
  Demux8/1 -> Scope8/1
  Demux6/3 -> Scope5/3
  Demux57/1 -> Scope57/1
  [V25abc] -> Demux30/1
  Demux65/2 -> Scope65/2
  Demux64/2 -> Scope64/2
  Demux2/2 -> Scope1/2
  [V22abc] -> Demux26/1
  [V5abc] -> Demux9/1
  Demux/2 -> Scope/2
  [I19abc] -> Demux19/1
  [I30abc] -> Demux57/1
  Demux4/2 -> Scope3/2
  Demux5/1 -> Scope4/1
  Demux23/1 -> Scope23/1
  Demux32/3 -> Scope32/3
  Demux58/2 -> Scope58/2
  Demux61/3 -> Scope61/3
  Demux2/1 -> Scope1/1
  Demux15/2 -> Scope15/2
  Demux9/1 -> Scope9/1
  [V7abc] -> Demux42/1
  Demux55/1 -> Scope55/1
  [V2abc] -> Demux1/1
  Demux43/2 -> Scope43/2
  Demux45/3 -> Scope45/3
  [I21abc] -> Demux25/1
  Demux7/2 -> Scope7/2
  [V4abc] -> Demux6/1
  Demux5/2 -> Scope4/2
  [V16abc] -> Demux12/1
  Demux41/1 -> Scope41/1
  Demux5/3 -> Scope4/3
  Demux19/1 -> Scope19/1
  [I26abc] -> Demux33/1
  Demux16/1 -> Scope16/1
  Demux8/3 -> Scope8/3
  Demux6/1 -> Scope5/1
  Demux3/1 -> Scope2/1
  [V18abc] -> Demux16/1
  Demux41/3 -> Scope41/3
  Demux3/3 -> Scope2/3
  Demux4/1 -> Scope3/1
  Demux7/1 -> Scope7/1
  [I33abc] -> Demux63/1
  [V9abc] -> Demux38/1
  Demux2/3 -> Scope1/3
  Demux8/2 -> Scope8/2
  [V1abc] -> Demux/1
  Demux1/1 -> Scope6/1
  Demux50/1 -> Scope50/1
  Demux21/1 -> Scope21/1
  [I31abc] -> Demux59/1
  Demux1/2 -> Scope6/2
  Demux49/2 -> Scope49/2
  Demux7/3 -> Scope7/3
  Demux3/2 -> Scope2/2
  [I2abc] -> Demux2/1
  [I17abc] -> Demux15/1
  Demux64/3 -> Scope64/3
  Demux62/2 -> Scope62/2
  connections:
  Three-Phase V-I Measurement28/RConn3 -- Three-Phase Parallel RLC Load23/LConn3 -- Three-Phase Series RLC Branch27/LConn3
  Load Flow Bus25/LConn1 -- Three-Phase V-I Measurement25/RConn1 -- Three-Phase Parallel RLC Load21/LConn1 -- Three-Phase Series RLC Branch25/LConn1
  Three-Phase Parallel RLC Load4/LConn2 -- Three-Phase Series RLC Branch5/LConn2 -- Three-Phase V-I Measurement3/RConn2 -- Three-Phase Series RLC Branch24/LConn2
  Load Flow Bus/LConn1 -- Three-Phase Parallel RLC Load6/LConn1 -- Three-Phase V-I Measurement17/RConn1
  Three-Phase Series RLC Branch16/LConn2 -- Three-Phase Parallel RLC Load7/LConn2 -- Three-Phase V-I Measurement16/RConn2
  Three-Phase V-I Measurement18/RConn3 -- Series RLC Branch39/LConn1 -- Series RLC Branch38/LConn1 -- Three-Phase Parallel RLC Load17/LConn3 -- Three-Phase Series RLC Branch17/LConn3
  Three-Phase Series RLC Branch10/LConn2 -- Three-Phase Parallel RLC Load13/LConn2 -- Three-Phase V-I Measurement10/RConn2
  Three-Phase Series RLC Branch15/LConn2 -- Three-Phase Parallel RLC Load8/LConn2 -- Three-Phase V-I Measurement15/RConn2
  Three-Phase V-I Measurement/RConn1 -- Three-Phase Series RLC Branch1/LConn1 -- Three-Phase Series RLC Branch23/LConn1 -- Load Flow Bus16/LConn1
  Load Flow Bus13/LConn1 -- Three-Phase Parallel RLC Load3/LConn1 -- Three-Phase V-I Measurement2/RConn1 -- Three-Phase Series RLC Branch4/LConn1
  Three-Phase Series RLC Branch2/LConn1 -- Load Flow Bus15/LConn1 -- Three-Phase V-I Measurement4/RConn1 -- Three-Phase Series RLC Branch22/LConn1 -- Three-Phase Parallel RLC Load1/LConn1
  Load Flow Bus4/LConn1 -- Three-Phase V-I Measurement13/RConn1 -- Three-Phase Series RLC Branch13/LConn1 -- Three-Phase Parallel RLC Load10/LConn1
  Three-Phase Series RLC Branch6/LConn2 -- Three-Phase Parallel RLC Load5/LConn2 -- Three-Phase V-I Measurement6/RConn2
  Three-Phase Parallel RLC Load23/LConn1 -- Load Flow Bus27/LConn1 -- Three-Phase V-I Measurement28/RConn1 -- Three-Phase Series RLC Branch27/LConn1
  Three-Phase Series RLC Branch13/LConn2 -- Three-Phase Parallel RLC Load10/LConn2 -- Three-Phase V-I Measurement13/RConn2
  Series RLC Branch28/LConn1 -- Three-Phase V-I Measurement12/RConn1 -- Load Flow Bus5/LConn1 -- Three-Phase Series RLC Branch12/LConn1 -- Three-Phase Parallel RLC Load11/LConn1 -- Series RLC Branch30/RConn1
  Load Flow Bus7/LConn1 -- Three-Phase Parallel RLC Load13/LConn1 -- Three-Phase V-I Measurement10/RConn1 -- Three-Phase Series RLC Branch10/LConn1
  Three-Phase V-I Measurement24/RConn3 -- Three-Phase Series RLC Branch21/LConn3 -- Three-Phase Parallel RLC Load31/LConn3
  Three-Phase Series RLC Branch8/LConn2 -- Three-Phase V-I Measurement8/RConn2 -- Three-Phase Parallel RLC Load15/LConn2
  Three-Phase V-I Measurement10/RConn3 -- Three-Phase Parallel RLC Load13/LConn3 -- Three-Phase Series RLC Branch10/LConn3
  Series RLC Branch18/RConn1 -- Three-Phase Series RLC Branch7/LConn1 -- Load Flow Bus10/LConn1 -- Three-Phase V-I Measurement7/RConn1 -- Three-Phase Parallel RLC Load16/LConn1 -- Series RLC Branch16/LConn1
  Three-Phase Parallel RLC Load24/LConn1 -- Load Flow Bus28/LConn1 -- Three-Phase V-I Measurement32/RConn1 -- Three-Phase Series RLC Branch28/LConn1
  Three-Phase V-I Measurement3/RConn3 -- Three-Phase Series RLC Branch5/LConn3 -- Three-Phase Parallel RLC Load4/LConn3 -- Three-Phase Series RLC Branch24/LConn3
  Three-Phase V-I Measurement11/RConn3 -- Three-Phase Parallel RLC Load12/LConn3 -- Three-Phase Series RLC Branch11/LConn3
  Three-Phase Series RLC Branch11/LConn1 -- Load Flow Bus6/LConn1 -- Three-Phase V-I Measurement11/RConn1 -- Three-Phase Parallel RLC Load12/LConn1
  Three-Phase Series RLC Branch19/LConn2 -- Three-Phase V-I Measurement21/RConn2 -- Three-Phase Parallel RLC Load29/LConn2
  Three-Phase V-I Measurement9/RConn1 -- Three-Phase Series RLC Branch9/LConn1 -- Load Flow Bus8/LConn1 -- Three-Phase Parallel RLC Load14/LConn1
  Three-Phase Parallel RLC Load4/LConn1 -- Load Flow Bus12/LConn1 -- Three-Phase V-I Measurement3/RConn1 -- Three-Phase Series RLC Branch24/LConn1 -- Three-Phase Series RLC Branch5/LConn1
  Three-Phase Series RLC Branch11/LConn2 -- Three-Phase Parallel RLC Load12/LConn2 -- Three-Phase V-I Measurement11/RConn2
  Three-Phase Series RLC Branch25/LConn2 -- Three-Phase Parallel RLC Load21/LConn2 -- Three-Phase V-I Measurement25/RConn2
  Three-Phase V-I Measurement25/RConn3 -- Three-Phase Parallel RLC Load21/LConn3 -- Three-Phase Series RLC Branch25/LConn3
  Three-Phase Parallel RLC Load25/LConn1 -- Load Flow Bus29/LConn1 -- Three-Phase V-I Measurement31/RConn1 -- Three-Phase Series RLC Branch29/LConn1
  Three-Phase Series RLC Branch22/LConn3 -- Three-Phase Series RLC Branch2/LConn3 -- Three-Phase Parallel RLC Load1/LConn3 -- Three-Phase V-I Measurement4/RConn3
  Three-Phase V-I Measurement13/RConn3 -- Three-Phase Parallel RLC Load10/LConn3 -- Three-Phase Series RLC Branch13/LConn3
  Three-Phase Parallel RLC Load29/LConn1 -- Load Flow Bus20/LConn1 -- Three-Phase V-I Measurement21/RConn1 -- Three-Phase Series RLC Branch19/LConn1
  Three-Phase V-I Measurement14/RConn2 -- Three-Phase Series RLC Branch14/LConn2 -- Three-Phase Parallel RLC Load9/LConn2
  Three-Phase V-I Measurement15/RConn3 -- Three-Phase Parallel RLC Load8/LConn3 -- Three-Phase Series RLC Branch15/LConn3
  Three-Phase V-I Measurement5/RConn3 -- Three-Phase Parallel RLC Load2/LConn3 -- Three-Phase Series RLC Branch3/LConn3
  Series RLC Branch17/LConn1 -- Three-Phase Parallel RLC Load16/LConn3 -- Three-Phase V-I Measurement7/RConn3 -- Three-Phase Series RLC Branch7/LConn3 -- Series RLC Branch18/LConn1
  Three-Phase Series RLC Branch26/LConn2 -- Three-Phase V-I Measurement26/RConn2 -- Three-Phase Parallel RLC Load22/LConn2
  Three-Phase V-I Measurement8/RConn3 -- Three-Phase Parallel RLC Load15/LConn3 -- Three-Phase Series RLC Branch8/LConn3
  Three-Phase Parallel RLC Load15/LConn1 -- Three-Phase V-I Measurement8/RConn1 -- Load Flow Bus9/LConn1 -- Three-Phase Series RLC Branch8/LConn1
  Three-Phase Series RLC Branch27/LConn2 -- Three-Phase Parallel RLC Load23/LConn2 -- Three-Phase V-I Measurement28/RConn2
  Three-Phase V-I Measurement21/RConn3 -- Three-Phase Parallel RLC Load29/LConn3 -- Three-Phase Series RLC Branch19/LConn3
  Three-Phase V-I Measurement1/RConn1 -- Load Flow Bus17/LConn1 -- Three-Phase Series RLC Branch/LConn1
  Series RLC Branch29/RConn1 -- Three-Phase V-I Measurement12/RConn2 -- Three-Phase Series RLC Branch12/LConn2 -- Three-Phase Parallel RLC Load11/LConn2 -- Series RLC Branch28/RConn1
  Three-Phase V-I Measurement2/RConn3 -- Three-Phase Parallel RLC Load3/LConn3 -- Three-Phase Series RLC Branch4/LConn3
  Three-Phase Series RLC Branch4/LConn2 -- Three-Phase Parallel RLC Load3/LConn2 -- Three-Phase V-I Measurement2/RConn2
  Series RLC Branch29/LConn1 -- Three-Phase V-I Measurement12/RConn3 -- Three-Phase Series RLC Branch12/LConn3 -- Three-Phase Parallel RLC Load11/LConn3 -- Series RLC Branch30/LConn1
  Load Flow Bus3/LConn1 -- Three-Phase Parallel RLC Load9/LConn1 -- Three-Phase V-I Measurement14/RConn1 -- Three-Phase Series RLC Branch14/LConn1
  Three-Phase Series RLC Branch9/LConn2 -- Three-Phase Parallel RLC Load14/LConn2 -- Three-Phase V-I Measurement9/RConn2
  Load Flow Bus14/LConn1 -- Three-Phase Parallel RLC Load2/LConn1 -- Three-Phase V-I Measurement5/RConn1 -- Three-Phase Series RLC Branch3/LConn1
  Three-Phase V-I Measurement6/RConn3 -- Three-Phase Parallel RLC Load5/LConn3 -- Three-Phase Series RLC Branch6/LConn3
  Load Flow Bus26/LConn1 -- Three-Phase V-I Measurement26/RConn1 -- Three-Phase Series RLC Branch26/LConn1 -- Three-Phase Parallel RLC Load22/LConn1
  Load Flow Bus2/LConn1 -- Three-Phase V-I Measurement15/RConn1 -- Three-Phase Parallel RLC Load8/LConn1 -- Three-Phase Series RLC Branch15/LConn1
  Three-Phase Series RLC Branch29/LConn2 -- Three-Phase Parallel RLC Load25/LConn2 -- Three-Phase V-I Measurement31/RConn2
  Three-Phase V-I Measurement31/RConn3 -- Three-Phase Parallel RLC Load25/LConn3 -- Three-Phase Series RLC Branch29/LConn3
  Load Flow Bus1/LConn1 -- Three-Phase V-I Measurement16/RConn1 -- Three-Phase Parallel RLC Load7/LConn1 -- Three-Phase Series RLC Branch16/LConn1
  Three-Phase Series RLC Branch28/LConn2 -- Three-Phase Parallel RLC Load24/LConn2 -- Three-Phase V-I Measurement32/RConn2
  Three-Phase V-I Measurement27/RConn1 -- Load Flow Bus32/LConn1 -- Three-Phase Parallel RLC Load27/LConn1
  Three-Phase V-I Measurement19/RConn3 -- Series RLC Branch44/LConn1 -- Series RLC Branch45/LConn1 -- Three-Phase Parallel RLC Load20/LConn3 -- Three-Phase Series RLC Branch18/LConn3
  Three-Phase V-I Measurement32/RConn3 -- Three-Phase Parallel RLC Load24/LConn3 -- Three-Phase Series RLC Branch28/LConn3
  Three-Phase V-I Measurement26/RConn3 -- Three-Phase Series RLC Branch26/LConn3 -- Three-Phase Parallel RLC Load22/LConn3
  Three-Phase V-I Measurement9/RConn3 -- Three-Phase Parallel RLC Load14/LConn3 -- Three-Phase Series RLC Branch9/LConn3
  Three-Phase Series RLC Branch3/LConn2 -- Three-Phase Parallel RLC Load2/LConn2 -- Three-Phase V-I Measurement5/RConn2
  Three-Phase Parallel RLC Load5/LConn1 -- Load Flow Bus11/LConn1 -- Three-Phase V-I Measurement6/RConn1 -- Three-Phase Series RLC Branch6/LConn1
  Three-Phase V-I Measurement16/RConn3 -- Three-Phase Parallel RLC Load7/LConn3 -- Three-Phase Series RLC Branch16/LConn3
  Three-Phase V-I Measurement4/RConn2 -- Three-Phase Parallel RLC Load1/LConn2 -- Three-Phase Series RLC Branch2/LConn2 -- Three-Phase Series RLC Branch22/LConn2
  Three-Phase Parallel RLC Load9/LConn3 -- Three-Phase Series RLC Branch14/LConn3 -- Three-Phase V-I Measurement14/RConn3
  Three-Phase Series RLC Branch21/RConn3 -- Three-Phase V-I Measurement23/LConn3
  Three-Phase Series RLC Branch11/RConn2 -- Three-Phase V-I Measurement12/LConn2
  Three-Phase Series RLC Branch24/RConn2 -- Three-Phase V-I Measurement25/LConn2
  Three-Phase V-I Measurement1/LConn2 -- Three-Phase Source/RConn2
  Three-Phase Series RLC Branch7/RConn1 -- Three-Phase V-I Measurement8/LConn1
  Three-Phase Series RLC Branch25/RConn3 -- Three-Phase V-I Measurement26/LConn3
  Three-Phase V-I Measurement1/RConn2 -- Three-Phase Series RLC Branch/LConn2
  Three-Phase Series RLC Branch12/RConn1 -- Three-Phase V-I Measurement13/LConn1
  Three-Phase Series RLC Branch5/RConn1 -- Three-Phase V-I Measurement6/LConn1
  Three-Phase V-I Measurement/RConn3 -- Three-Phase Series RLC Branch23/LConn3 -- Three-Phase Series RLC Branch1/LConn3
  Three-Phase V-I Measurement2/LConn2 -- Three-Phase Series RLC Branch3/RConn2
  Three-Phase V-I Measurement17/RConn2 -- Three-Phase Parallel RLC Load6/LConn2
  Three-Phase Series RLC Branch27/RConn1 -- Three-Phase V-I Measurement32/LConn1
  Three-Phase V-I Measurement10/LConn2 -- Three-Phase Series RLC Branch9/RConn2
  Three-Phase Series RLC Branch22/RConn2 -- Three-Phase V-I Measurement22/LConn2
  Three-Phase Series RLC Branch5/RConn3 -- Three-Phase V-I Measurement6/LConn3
  Three-Phase Series RLC Branch16/RConn3 -- Three-Phase V-I Measurement17/LConn3
  Three-Phase Series RLC Branch4/RConn1 -- Three-Phase V-I Measurement3/LConn1
  Three-Phase V-I Measurement23/RConn3 -- Series RLC Branch36/LConn1 -- Series RLC Branch35/LConn1 -- Three-Phase Parallel RLC Load19/LConn3
  Three-Phase Series RLC Branch12/RConn3 -- Three-Phase V-I Measurement13/LConn3
  Three-Phase Series RLC Branch3/RConn1 -- Three-Phase V-I Measurement2/LConn1
  Three-Phase V-I Measurement19/LConn2 -- Three-Phase Series RLC Branch17/RConn2
  Three-Phase Series RLC Branch18/RConn1 -- Three-Phase V-I Measurement21/LConn1
  Three-Phase Series RLC Branch9/RConn3 -- Three-Phase V-I Measurement10/LConn3
  Three-Phase Series RLC Branch6/RConn3 -- Three-Phase V-I Measurement7/LConn3
  Three-Phase Series RLC Branch23/RConn1 -- Three-Phase V-I Measurement18/LConn1
  Three-Phase V-I Measurement16/LConn2 -- Three-Phase Series RLC Branch15/RConn2
  Three-Phase Series RLC Branch21/RConn1 -- Three-Phase V-I Measurement23/LConn1
  Three-Phase Series RLC Branch28/RConn3 -- Three-Phase V-I Measurement31/LConn3
  Three-Phase Series RLC Branch24/RConn3 -- Three-Phase V-I Measurement25/LConn3
  Three-Phase V-I Measurement4/LConn2 -- Three-Phase Series RLC Branch1/RConn2
  Three-Phase V-I Measurement14/LConn2 -- Three-Phase Series RLC Branch13/RConn2
  Three-Phase Series RLC Branch3/RConn3 -- Three-Phase V-I Measurement2/LConn3
  Three-Phase V-I Measurement17/LConn2 -- Three-Phase Series RLC Branch16/RConn2
  Three-Phase V-I Measurement1/RConn3 -- Three-Phase Series RLC Branch/LConn3
  Three-Phase Series RLC Branch20/RConn3 -- Three-Phase V-I Measurement24/LConn3
  Three-Phase V-I Measurement27/RConn3 -- Three-Phase Parallel RLC Load27/LConn3
  Three-Phase Series RLC Branch27/RConn2 -- Three-Phase V-I Measurement32/LConn2
  Three-Phase V-I Measurement1/LConn3 -- Three-Phase Source/RConn3
  Three-Phase Series RLC Branch29/RConn1 -- Three-Phase V-I Measurement29/LConn1
  Three-Phase Series RLC Branch4/RConn3 -- Three-Phase V-I Measurement3/LConn3
  Three-Phase Series RLC Branch14/RConn1 -- Three-Phase V-I Measurement15/LConn1
  Three-Phase Series RLC Branch/RConn3 -- Three-Phase V-I Measurement/LConn3
  Three-Phase V-I Measurement29/LConn2 -- Three-Phase Series RLC Branch29/RConn2
  Three-Phase Series RLC Branch9/RConn1 -- Three-Phase V-I Measurement10/LConn1
  Three-Phase Series RLC Branch23/RConn2 -- Three-Phase V-I Measurement18/LConn2
  Three-Phase V-I Measurement9/LConn2 -- Three-Phase Series RLC Branch8/RConn2
  Three-Phase V-I Measurement7/LConn2 -- Three-Phase Series RLC Branch6/RConn2
  Three-Phase Series RLC Branch26/RConn1 -- Three-Phase V-I Measurement28/LConn1
  Three-Phase Series RLC Branch16/RConn1 -- Three-Phase V-I Measurement17/LConn1
  Three-Phase V-I Measurement21/LConn2 -- Three-Phase Series RLC Branch18/RConn2
  Three-Phase V-I Measurement27/LConn2 -- Three-Phase Series RLC Branch31/RConn2
  Three-Phase V-I Measurement1/LConn1 -- Three-Phase Source/RConn1
  Three-Phase V-I Measurement8/LConn2 -- Three-Phase Series RLC Branch7/RConn2
  Three-Phase Series RLC Branch13/RConn3 -- Three-Phase V-I Measurement14/LConn3
  Three-Phase V-I Measurement17/RConn3 -- Three-Phase Parallel RLC Load6/LConn3
  Three-Phase Series RLC Branch1/RConn3 -- Three-Phase V-I Measurement4/LConn3
  Three-Phase Series RLC Branch2/RConn1 -- Three-Phase V-I Measurement5/LConn1
  Three-Phase Series RLC Branch25/RConn1 -- Three-Phase V-I Measurement26/LConn1
  Three-Phase Series RLC Branch28/RConn1 -- Three-Phase V-I Measurement31/LConn1
  Three-Phase Series RLC Branch24/RConn1 -- Three-Phase V-I Measurement25/LConn1
  Three-Phase V-I Measurement15/LConn2 -- Three-Phase Series RLC Branch14/RConn2
  Three-Phase Series RLC Branch2/RConn3 -- Three-Phase V-I Measurement5/LConn3
  Three-Phase Series RLC Branch10/RConn3 -- Three-Phase V-I Measurement11/LConn3
  Three-Phase Series RLC Branch8/RConn3 -- Three-Phase V-I Measurement9/LConn3
  Three-Phase Series RLC Branch27/RConn3 -- Three-Phase V-I Measurement32/LConn3
  Three-Phase V-I Measurement6/LConn2 -- Three-Phase Series RLC Branch5/RConn2
  Three-Phase Series RLC Branch21/RConn2 -- Three-Phase V-I Measurement23/LConn2
  Three-Phase Series RLC Branch8/RConn1 -- Three-Phase V-I Measurement9/LConn1
  Three-Phase Series RLC Branch19/RConn3 -- Three-Phase V-I Measurement20/LConn3
  Three-Phase Series RLC Branch29/RConn3 -- Three-Phase V-I Measurement29/LConn3
  Three-Phase Series RLC Branch6/RConn1 -- Three-Phase V-I Measurement7/LConn1
  Three-Phase V-I Measurement3/LConn2 -- Three-Phase Series RLC Branch4/RConn2
  Three-Phase Series RLC Branch19/RConn1 -- Three-Phase V-I Measurement20/LConn1
  Three-Phase Series RLC Branch26/RConn3 -- Three-Phase V-I Measurement28/LConn3
  Three-Phase Series RLC Branch23/RConn3 -- Three-Phase V-I Measurement18/LConn3
  Three-Phase Series RLC Branch/RConn1 -- Three-Phase V-I Measurement/LConn1
  Three-Phase Series RLC Branch1/LConn2 -- Three-Phase V-I Measurement/RConn2 -- Three-Phase Series RLC Branch23/LConn2
  Three-Phase Series RLC Branch14/RConn3 -- Three-Phase V-I Measurement15/LConn3
  Three-Phase Series RLC Branch22/RConn3 -- Three-Phase V-I Measurement22/LConn3
  Three-Phase Series RLC Branch15/RConn1 -- Three-Phase V-I Measurement16/LConn1
  Three-Phase Series RLC Branch18/RConn3 -- Three-Phase V-I Measurement21/LConn3
  Three-Phase V-I Measurement/LConn2 -- Three-Phase Series RLC Branch/RConn2
  Three-Phase Series RLC Branch1/RConn1 -- Three-Phase V-I Measurement4/LConn1
  Three-Phase V-I Measurement26/LConn2 -- Three-Phase Series RLC Branch25/RConn2
  Three-Phase Series RLC Branch17/RConn1 -- Three-Phase V-I Measurement19/LConn1
  Three-Phase Series RLC Branch22/RConn1 -- Three-Phase V-I Measurement22/LConn1
  Three-Phase Series RLC Branch11/RConn3 -- Three-Phase V-I Measurement12/LConn3
  Three-Phase Series RLC Branch11/RConn1 -- Three-Phase V-I Measurement12/LConn1
  Three-Phase Series RLC Branch17/RConn3 -- Three-Phase V-I Measurement19/LConn3
  Three-Phase Series RLC Branch20/RConn1 -- Three-Phase V-I Measurement24/LConn1
  Three-Phase Series RLC Branch15/RConn3 -- Three-Phase V-I Measurement16/LConn3
  Three-Phase V-I Measurement11/LConn2 -- Three-Phase Series RLC Branch10/RConn2
  Three-Phase Series RLC Branch10/RConn1 -- Three-Phase V-I Measurement11/LConn1
  Three-Phase Series RLC Branch31/RConn1 -- Three-Phase V-I Measurement27/LConn1
  Three-Phase V-I Measurement5/LConn2 -- Three-Phase Series RLC Branch2/RConn2
  Three-Phase V-I Measurement13/LConn2 -- Three-Phase Series RLC Branch12/RConn2
  Three-Phase Series RLC Branch26/RConn2 -- Three-Phase V-I Measurement28/LConn2
  Three-Phase V-I Measurement31/LConn2 -- Three-Phase Series RLC Branch28/RConn2
  Three-Phase V-I Measurement20/LConn2 -- Three-Phase Series RLC Branch19/RConn2
  Three-Phase Series RLC Branch20/RConn2 -- Three-Phase V-I Measurement24/LConn2
  Three-Phase Series RLC Branch13/RConn1 -- Three-Phase V-I Measurement14/LConn1
  Three-Phase Series RLC Branch7/RConn3 -- Three-Phase V-I Measurement8/LConn3
  Three-Phase V-I Measurement30/LConn2 -- Three-Phase Series RLC Branch30/RConn2
  Three-Phase V-I Measurement30/LConn3 -- Three-Phase Series RLC Branch30/RConn3
  Three-Phase V-I Measurement30/LConn1 -- Three-Phase Series RLC Branch30/RConn1
  Series RLC Branch4/LConn1 -- Series RLC Branch3/LConn1 -- Ground/LConn1 -- Series RLC Branch2/LConn1
  Three-Phase V-I Measurement27/LConn3 -- Three-Phase Series RLC Branch31/RConn3
  Series RLC Branch7/RConn1 -- Series RLC Branch8/RConn1 -- Ground2/LConn1 -- Series RLC Branch9/RConn1
  Series RLC Branch15/RConn1 -- Series RLC Branch13/LConn1
  Series RLC Branch13/RConn1 -- Series RLC Branch14/RConn1
  Series RLC Branch14/LConn1 -- Series RLC Branch15/LConn1
  Series RLC Branch16/RConn1 -- Three-Phase Series RLC Branch7/LConn2 -- Three-Phase V-I Measurement7/RConn2 -- Three-Phase Parallel RLC Load16/LConn2 -- Series RLC Branch17/RConn1
  Three-Phase V-I Measurement24/RConn2 -- Three-Phase Series RLC Branch21/LConn2 -- Three-Phase Parallel RLC Load31/LConn2
  Three-Phase Series RLC Branch21/LConn1 -- Load Flow Bus23/LConn1 -- Three-Phase V-I Measurement24/RConn1 -- Three-Phase Parallel RLC Load31/LConn1
  Three-Phase V-I Measurement22/RConn1 -- Load Flow Bus22/LConn1 -- Three-Phase Parallel RLC Load18/LConn1 -- Three-Phase Series RLC Branch20/LConn1
  Three-Phase V-I Measurement22/RConn2 -- Three-Phase Parallel RLC Load18/LConn2 -- Three-Phase Series RLC Branch20/LConn2
  Three-Phase V-I Measurement22/RConn3 -- Three-Phase Parallel RLC Load18/LConn3 -- Three-Phase Series RLC Branch20/LConn3
  Series RLC Branch26/RConn1 -- Series RLC Branch25/RConn1
  Series RLC Branch27/LConn1 -- Series RLC Branch26/LConn1
  Series RLC Branch25/LConn1 -- Series RLC Branch27/RConn1
  Three-Phase V-I Measurement27/RConn2 -- Three-Phase Parallel RLC Load27/LConn2
  Three-Phase V-I Measurement30/RConn3 -- Series RLC Branch33/LConn1 -- Series RLC Branch32/LConn1 -- Three-Phase Parallel RLC Load26/LConn3 -- Three-Phase Series RLC Branch31/LConn3
  Three-Phase V-I Measurement29/RConn1 -- Series RLC Branch12/RConn1 -- Series RLC Branch10/LConn1 -- Three-Phase Parallel RLC Load28/LConn1 -- Three-Phase Series RLC Branch30/LConn1 -- Load Flow Bus30/LConn1
  Three-Phase V-I Measurement20/RConn3 -- Three-Phase Parallel RLC Load30/LConn3 -- Series RLC Branch41/LConn1 -- Series RLC Branch42/LConn1
  Three-Phase V-I Measurement20/RConn1 -- Load Flow Bus21/LConn1 -- Series RLC Branch42/RConn1 -- Series RLC Branch40/LConn1 -- Three-Phase Parallel RLC Load30/LConn1
  Three-Phase V-I Measurement20/RConn2 -- Series RLC Branch40/RConn1 -- Series RLC Branch41/RConn1 -- Three-Phase Parallel RLC Load30/LConn2
  Three-Phase Series RLC Branch18/LConn2 -- Series RLC Branch43/RConn1 -- Series RLC Branch44/RConn1 -- Three-Phase Parallel RLC Load20/LConn2 -- Three-Phase V-I Measurement19/RConn2
  Three-Phase Parallel RLC Load20/LConn1 -- Series RLC Branch45/RConn1 -- Series RLC Branch43/LConn1 -- Load Flow Bus19/LConn1 -- Three-Phase V-I Measurement19/RConn1 -- Three-Phase Series RLC Branch18/LConn1
  Three-Phase Series RLC Branch17/LConn2 -- Three-Phase Parallel RLC Load17/LConn2 -- Series RLC Branch37/RConn1 -- Series RLC Branch38/RConn1 -- Three-Phase V-I Measurement18/RConn2
  Three-Phase Parallel RLC Load17/LConn1 -- Series RLC Branch39/RConn1 -- Series RLC Branch37/LConn1 -- Load Flow Bus18/LConn1 -- Three-Phase Series RLC Branch17/LConn1 -- Three-Phase V-I Measurement18/RConn1
  Three-Phase V-I Measurement23/RConn2 -- Three-Phase Parallel RLC Load19/LConn2 -- Series RLC Branch34/RConn1 -- Series RLC Branch35/RConn1
  Three-Phase Parallel RLC Load19/LConn1 -- Series RLC Branch36/RConn1 -- Series RLC Branch34/LConn1 -- Load Flow Bus24/LConn1 -- Three-Phase V-I Measurement23/RConn1
  Three-Phase Parallel RLC Load26/LConn2 -- Series RLC Branch31/RConn1 -- Series RLC Branch32/RConn1 -- Three-Phase Series RLC Branch31/LConn2 -- Three-Phase V-I Measurement30/RConn2
  Three-Phase V-I Measurement30/RConn1 -- Three-Phase Parallel RLC Load26/LConn1 -- Series RLC Branch33/RConn1 -- Series RLC Branch31/LConn1 -- Load Flow Bus31/LConn1 -- Three-Phase Series RLC Branch31/LConn1
  Three-Phase V-I Measurement29/RConn3 -- Three-Phase Parallel RLC Load28/LConn3 -- Series RLC Branch11/LConn1 -- Series RLC Branch12/LConn1 -- Three-Phase Series RLC Branch30/LConn3
  Three-Phase Parallel RLC Load28/LConn2 -- Series RLC Branch10/RConn1 -- Series RLC Branch11/RConn1 -- Three-Phase Series RLC Branch30/LConn2 -- Three-Phase V-I Measurement29/RConn2
